simulink model "SWC_FDC_type"  (R2021b)
settings: Solver=FixedStepDiscrete  StartTime=0.0  StopTime=10.0  FixedStep=0.001  RelTol=1e-3
values from neighbouring files (symbols this model uses):
  C_TASK_5MS_S = (	C_TICK_TIME_S      	)    [vcu_local_hdr.m]
  DID_VCUKey = uint16(0x0202)    [vcu_local_hdr.m]
  DID_XWD = uint16(513)    [vcu_local_hdr.m]
  DIDLen_DKCKey = uint16(8)    [vcu_local_hdr.m]
  DIDLen_FoxPiBattSta = uint16(4)    [vcu_local_hdr.m]
  DIDLen_FoxPiBrakeSta = uint16(13)    [vcu_local_hdr.m]
  DIDLen_FoxPiButtonSta = uint16(2)    [vcu_local_hdr.m]
  DIDLen_FoxPiCtrlEnSw = uint16(1)    [vcu_local_hdr.m]
  DIDLen_FoxPiDrivingCtrl = uint16(21)    [vcu_local_hdr.m]
  DIDLen_FoxPiEPSSta = uint16(11)    [vcu_local_hdr.m]
  DIDLen_FoxPiLampCtrl = uint16(6)    [vcu_local_hdr.m]
  DIDLen_FoxPiLampSta = uint16(2)    [vcu_local_hdr.m]
  DIDLen_FoxPiMotionSta = uint16(13)    [vcu_local_hdr.m]
  DIDLen_FoxPiMotorSta = uint16(11)    [vcu_local_hdr.m]
  DIDLen_FoxPiPedalPos = uint16(3)    [vcu_local_hdr.m]
  DIDLen_FoxPiPTGUSSSw = uint16(1)    [vcu_local_hdr.m]
  DIDLen_FoxPiShifterAllow = uint16(3)    [vcu_local_hdr.m]
  DIDLen_FoxPiSwSta = uint16(2)    [vcu_local_hdr.m]
  DIDLen_FoxPiTPMSSta = uint16(13)    [vcu_local_hdr.m]
  DIDLen_FoxPiUSSDist = uint16(20)    [vcu_local_hdr.m]
  DIDLen_FoxPiUSSFaultSta = uint16(2)    [vcu_local_hdr.m]
  DIDLen_FoxPiWheelSpd = uint16(16)    [vcu_local_hdr.m]
  DIDNum_DKCKey = uint16(0x0202)    [vcu_local_hdr.m]
  DIDNum_FoxPiBattSta = uint16(0x100D)    [vcu_local_hdr.m]
  DIDNum_FoxPiBrakeSta = uint16(0x1003)    [vcu_local_hdr.m]
  DIDNum_FoxPiButtonSta = uint16(0x1006)    [vcu_local_hdr.m]
  DIDNum_FoxPiCtrlEnSw = uint16(0x1012)    [vcu_local_hdr.m]
  DIDNum_FoxPiDrivingCtrl = uint16(0x1001)    [vcu_local_hdr.m]
  DIDNum_FoxPiEPSSta = uint16(0x1005)    [vcu_local_hdr.m]
  DIDNum_FoxPiLampCtrl = uint16(0x100C)    [vcu_local_hdr.m]
  DIDNum_FoxPiLampSta = uint16(0x100B)    [vcu_local_hdr.m]
  DIDNum_FoxPiMotionSta = uint16(0x1002)    [vcu_local_hdr.m]
  DIDNum_FoxPiMotorSta = uint16(0x1010)    [vcu_local_hdr.m]
  DIDNum_FoxPiPedalPos = uint16(0x100F)    [vcu_local_hdr.m]
  DIDNum_FoxPiPTGUSSSw = uint16(0x1009)    [vcu_local_hdr.m]
  DIDNum_FoxPiShifterAllow = uint16(0x1011)    [vcu_local_hdr.m]
  DIDNum_FoxPiSwSta = uint16(0x100A)    [vcu_local_hdr.m]
  DIDNum_FoxPiTPMSSta = uint16(0x100E)    [vcu_local_hdr.m]
  DIDNum_FoxPiUSSDist = uint16(0x1007)    [vcu_local_hdr.m]
  DIDNum_FoxPiUSSFaultSta = uint16(0x1008)    [vcu_local_hdr.m]
  DIDNum_FoxPiWheelSpd = uint16(0x1004)    [vcu_local_hdr.m]
  DIDVCUKeyLength = uint16(8)    [vcu_local_hdr.m]
  DTC_10020B = Simulink.Parameter    [DTC_Constant_Definition.m]
  DTC_10020C = Simulink.Parameter    [DTC_Constant_Definition.m]
  DTC_10020D = Simulink.Parameter    [DTC_Constant_Definition.m]
  DTC_10020E = Simulink.Parameter    [DTC_Constant_Definition.m]
  DTC_100210 = Simulink.Parameter    [DTC_Constant_Definition.m]
  DTC_100211 = Simulink.Parameter    [DTC_Constant_Definition.m]
  DTC_100212 = Simulink.Parameter    [DTC_Constant_Definition.m]
  DTC_100213 = Simulink.Parameter    [DTC_Constant_Definition.m]
  DTC_100214 = Simulink.Parameter    [DTC_Constant_Definition.m]
  DTC_100215 = Simulink.Parameter    [DTC_Constant_Definition.m]
  DTC_100216 = Simulink.Parameter    [DTC_Constant_Definition.m]
  DTC_100217 = Simulink.Parameter    [DTC_Constant_Definition.m]
  DTC_100218 = Simulink.Parameter    [DTC_Constant_Definition.m]
  DTC_100219 = Simulink.Parameter    [DTC_Constant_Definition.m]
  DTC_10021A = Simulink.Parameter    [DTC_Constant_Definition.m]
  DTC_10021B = Simulink.Parameter    [DTC_Constant_Definition.m]
  DTC_10021C = Simulink.Parameter    [DTC_Constant_Definition.m]
  DTC_10021D = Simulink.Parameter    [DTC_Constant_Definition.m]
  DTC_10021E = Simulink.Parameter    [DTC_Constant_Definition.m]
  DTC_100220 = Simulink.Parameter    [DTC_Constant_Definition.m]
  DTC_100221 = Simulink.Parameter    [DTC_Constant_Definition.m]
  DTC_100223 = Simulink.Parameter    [DTC_Constant_Definition.m]
  DTC_100224 = Simulink.Parameter    [DTC_Constant_Definition.m]
  DTC_100225 = Simulink.Parameter    [DTC_Constant_Definition.m]
  DTC_100226 = Simulink.Parameter    [DTC_Constant_Definition.m]
  DTC_100227 = Simulink.Parameter    [DTC_Constant_Definition.m]
  DTC_100242 = Simulink.Parameter    [DTC_Constant_Definition.m]
  DTC_100243 = Simulink.Parameter    [DTC_Constant_Definition.m]
  DTC_100244 = Simulink.Parameter    [DTC_Constant_Definition.m]
  DTC_100247 = Simulink.Parameter    [DTC_Constant_Definition.m]
  DTC_100248 = Simulink.Parameter    [DTC_Constant_Definition.m]
  DTC_100249 = Simulink.Parameter    [DTC_Constant_Definition.m]
  DTC_100250 = Simulink.Parameter    [DTC_Constant_Definition.m]
  DTC_100251 = Simulink.Parameter    [DTC_Constant_Definition.m]
  DTC_100252 = Simulink.Parameter    [DTC_Constant_Definition.m]
  DTC_100A10 = Simulink.Parameter    [DTC_Constant_Definition.m]
  DTC_100A12 = Simulink.Parameter    [DTC_Constant_Definition.m]
  DTC_100A16 = Simulink.Parameter    [DTC_Constant_Definition.m]
  DTC_100A17 = Simulink.Parameter    [DTC_Constant_Definition.m]
  DTC_100A18 = Simulink.Parameter    [DTC_Constant_Definition.m]
  DTC_100A19 = Simulink.Parameter    [DTC_Constant_Definition.m]
  DTC_500B01 = Simulink.Parameter    [DTC_Constant_Definition.m]
  DTC_500B02 = Simulink.Parameter    [DTC_Constant_Definition.m]
  DTC_500B03 = Simulink.Parameter    [DTC_Constant_Definition.m]
  DTC_500B04 = Simulink.Parameter    [DTC_Constant_Definition.m]
  DTC_500B05 = Simulink.Parameter    [DTC_Constant_Definition.m]
  DTC_500B06 = Simulink.Parameter    [DTC_Constant_Definition.m]
  DTC_500B07 = Simulink.Parameter    [DTC_Constant_Definition.m]
  DTC_500B08 = Simulink.Parameter    [DTC_Constant_Definition.m]
  DTC_500B09 = Simulink.Parameter    [DTC_Constant_Definition.m]
  DTC_500B0A = Simulink.Parameter    [DTC_Constant_Definition.m]
  DTC_500B0B = Simulink.Parameter    [DTC_Constant_Definition.m]
  DTC_500B0C = Simulink.Parameter    [DTC_Constant_Definition.m]
  DTC_500B0D = Simulink.Parameter    [DTC_Constant_Definition.m]
  DTC_500B0E = Simulink.Parameter    [DTC_Constant_Definition.m]
  DTC_500B0F = Simulink.Parameter    [DTC_Constant_Definition.m]
  DTC_500B10 = Simulink.Parameter    [DTC_Constant_Definition.m]
  DTC_90021F = Simulink.Parameter    [DTC_Constant_Definition.m]
  DTC_90022F = Simulink.Parameter    [DTC_Constant_Definition.m]
  DTC_900253 = Simulink.Parameter    [DTC_Constant_Definition.m]
  DTC_900254 = Simulink.Parameter    [DTC_Constant_Definition.m]
  DTC_900301 = Simulink.Parameter    [DTC_Constant_Definition.m]
  DTC_900302 = Simulink.Parameter    [DTC_Constant_Definition.m]
  DTC_900303 = Simulink.Parameter    [DTC_Constant_Definition.m]
  DTC_900304 = Simulink.Parameter    [DTC_Constant_Definition.m]
  DTC_900305 = Simulink.Parameter    [DTC_Constant_Definition.m]
  DTC_900909 = Simulink.Parameter    [DTC_Constant_Definition.m]
  DTC_90090A = Simulink.Parameter    [DTC_Constant_Definition.m]
  DTC_90090B = Simulink.Parameter    [DTC_Constant_Definition.m]
  DTC_90090C = Simulink.Parameter    [DTC_Constant_Definition.m]
  DTC_90090D = Simulink.Parameter    [DTC_Constant_Definition.m]
  DTC_90090E = Simulink.Parameter    [DTC_Constant_Definition.m]
  DTC_90090F = Simulink.Parameter    [DTC_Constant_Definition.m]
  DTC_900910 = Simulink.Parameter    [DTC_Constant_Definition.m]
  DTC_900911 = Simulink.Parameter    [DTC_Constant_Definition.m]
  DTC_900912 = Simulink.Parameter    [DTC_Constant_Definition.m]
  DTC_900913 = Simulink.Parameter    [DTC_Constant_Definition.m]
  DTC_900914 = Simulink.Parameter    [DTC_Constant_Definition.m]
  ... (+54 more)
undefined symbols (not defined in the file or in its folder): f32_ApsOutVehSpdSig, KHAL_CANBusOffDebounce_cnt, KHAL_CANBusOffDebounce_s, KHAL_DKCDecryptEnable_flg_ovrdflg, KHAL_DKCDecryptEnable_flg_ovrdval, KHAL_RandomNumberY1_enum, KHAL_RandomNumberY2_enum, KHAL_RandomNumberY_ovrdflg, KHAL_TPMSRESBUTT_flg_ovrdflg, KHAL_TPMSRESBUTT_flg_ovrdval, KINP_ReadVinCode_flg, P_boolean, R_DIDWriteCDD_CSOP_DIDSet_DKCKey, R_DIDWriteCDD_CSOP_DIDSet_FoxPiBattSta, R_DIDWriteCDD_CSOP_DIDSet_FoxPiBrakeSta, R_DIDWriteCDD_CSOP_DIDSet_FoxPiButtonSta, R_DIDWriteCDD_CSOP_DIDSet_FoxPiCtrlEnSw, R_DIDWriteCDD_CSOP_DIDSet_FoxPiDrivingCtrl, R_DIDWriteCDD_CSOP_DIDSet_FoxPiEPSSta, R_DIDWriteCDD_CSOP_DIDSet_FoxPiLampCtrl, R_DIDWriteCDD_CSOP_DIDSet_FoxPiLampSta, R_DIDWriteCDD_CSOP_DIDSet_FoxPiMotionSta, R_DIDWriteCDD_CSOP_DIDSet_FoxPiMotorSta, R_DIDWriteCDD_CSOP_DIDSet_FoxPiPedalPos, R_DIDWriteCDD_CSOP_DIDSet_FoxPiPTGUSSSw, R_DIDWriteCDD_CSOP_DIDSet_FoxPiShifterAllow, R_DIDWriteCDD_CSOP_DIDSet_FoxPiSwSta, R_DIDWriteCDD_CSOP_DIDSet_FoxPiTPMSSta, R_DIDWriteCDD_CSOP_DIDSet_FoxPiUSSDist, R_DIDWriteCDD_CSOP_DIDSet_FoxPiUSSFaultSta, R_DIDWriteCDD_CSOP_DIDSet_FoxPiWheelSpd, R_E2E_CAN3_VCU1_CSOP_Write_CAN3_VCU1, R_E2E_CAN3_VCU1_toNIDEC_CSOP_Write_CAN3_VCU1_toNIDEC, R_E2E_CAN4_VCU1_CSOP_Write_CAN4_VCU1, R_FDCCDD_Inner_CSOP_FDC_AppCallSleep, R_HALIN_IMU_CSOP_IMUSetSta, R_HALINCDD_CSOP_PAS_Handler, R_HALINCDD_CSOP_ResetPedalZeroPosDone, R_HALINCDD_CSOP_TPMSSensorIDRegSetResults, R_HALINCDD_CSOP_UDS_Main, R_HALOUT_APS_CSOP_ApsOutput, R_HALOUTCDD_CSOP_AppNmStateReq, R_HALOUTCDD_CSOP_IVIReset, R_HALOUTCDD_CSOP_SetAcoreRebootCmdACK, R_HALOUTCDD_CSOP_SetSysPwrStat ... (+80)
libraries: FVT_lib x447, simulink x289, hcu_lib x19, hdlsllib x9, app x1, halin x1, halout x1, matrix_library x1, inp x1, outp x1
(part 7 of 15)

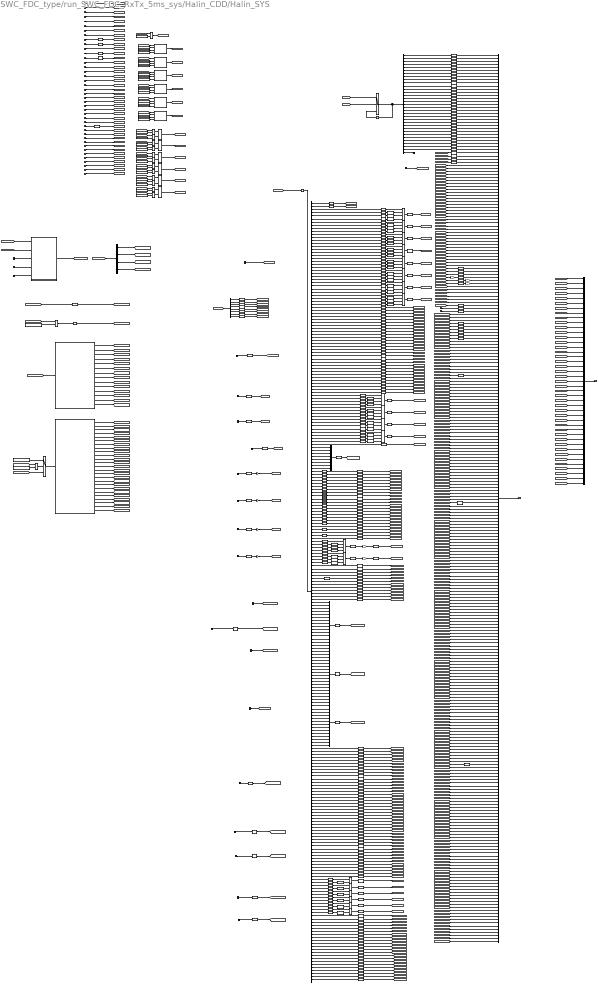
== system SWC_FDC_type/run_SWC_FDC_RxTx_5ms_sys/Halin_CDD/Halin_SYS ==
  note: Foxtron Pi
  note: CAN Bus Error
  note: CAN bus off debounce
  note: DID APS
  note: DID VCUKey
  note: DID BCM
  note: DID XWD
  GetSWID_status : Inport
  GetSWID_data : Inport  Port=2
  VHAL_AnyNMID_flg : Inport  Port=3
  VHAL_CurrentNmState_enum : Inport  Port=4
  VHAL_PwrReq_OTA_enum : Inport  Port=5
  VHAL_AllowMovThd_OTA_enum : Inport  Port=6
  VHAL_EvccAplusPwrUpReq_flg : Inport  Port=7
  VHAL_AcoreReadyToSlp_flg : Inport  Port=8
  VHAL_DidXWDSta_flg : Inport  Port=9
  VHAL_DidXWDData_enum : Inport  Port=10
  HAL_NvmReadData_raw : Inport  Port=11
  VHAL_DIDVCUKeyReadSta_flg : Inport  Port=12
  VHAL_GetDIDVCUKey_enum : Inport  Port=13
  VHAL_NvmProtectSta_flg : Inport  Port=14
  VHAL_AuxBattVolmV_100mV : Inport  Port=15
  VHAL_Pedal1Ref5V_raw : Inport  Port=16
  VHAL_Pedal2Ref5V_raw : Inport  Port=17
  VHAL_NetworkReqCalled_flg : Inport  Port=18
  VHAL_PmicBootReason_enum : Inport  Port=19
  VHAL_WisrBootReason_raw32 : Inport  Port=20
  BHAL_DIDGetData_raw : Inport  Port=21
  VHAL_AcoreRebootCmd_raw : Inport  Port=22
  VHAL_CAN1BusOff_raw : Inport  Port=23
  VHAL_CAN2BusOff_raw : Inport  Port=24
  VHAL_CAN3BusOff_raw : Inport  Port=25
  VHAL_CAN4BusOff_raw : Inport  Port=26
  VHAL_CAN5BusOff_raw : Inport  Port=27
  VHAL_CAN6BusOff_raw : Inport  Port=28
  VHAL_TPMSSensorIDRegSta_raw : Inport  Port=29
  VHAL_ResetPedalZeroPosReq_raw : Inport  Port=30
  VHAL_PmicBootPath_raw32 : Inport  Port=31
  VHAL_CAN1RxErrorCount_raw : Inport  Port=32
  VHAL_CAN1TxErrorCount_raw : Inport  Port=33
  VHAL_CAN2RxErrorCount_raw : Inport  Port=34
  VHAL_CAN2TxErrorCount_raw : Inport  Port=35
  VHAL_CAN3RxErrorCount_raw : Inport  Port=36
  VHAL_CAN3TxErrorCount_raw : Inport  Port=37
  VHAL_CAN4RxErrorCount_raw : Inport  Port=38
  VHAL_CAN4TxErrorCount_raw : Inport  Port=39
  VHAL_CAN5RxErrorCount_raw : Inport  Port=40
  VHAL_CAN5TxErrorCount_raw : Inport  Port=41
  VHAL_CAN6RxErrorCount_raw : Inport  Port=42
  VHAL_CAN6TxErrorCount_raw : Inport  Port=43
  AND : Logic  Inputs=1  AllPortsSameDT=off  OutDataTypeStr=boolean
  Bitwise OR{1..14} (14 alike) : simulink/Logic and Bit Operations/Bitwise Operator  logicop=OR  UseBitMask=off  NumInputPorts=4  BitMask=bin2dec('00000000000000000000')  BitMaskRealWorld=Stored Integer
  Bitwise OR{15..20} (6 alike) : simulink/Logic and Bit Operations/Bitwise Operator  logicop=OR  UseBitMask=off  NumInputPorts=2  BitMask=bin2dec('00000000000000000000')  BitMaskRealWorld=Stored Integer
  Bus Creator : BusCreator  Inputs=292  OutDataTypeStr=Bus: BHAL_SYS_outputs  NonVirtualBus=on
  Bus Creator4 : BusCreator  Inputs=43
  Bus Selector : BusSelector  OutputSignals=VHAL_DIDGetDKCKey_raw8,VHAL_DIDGetFoxPiDrivingCtrl_raw8,VHAL_DIDGetFoxPiLampCtrl_raw8,VHAL_DIDGetFoxPiCtrlEnSw_raw8
  Constant{,74..85} (13 alike) : Constant  Value=ZERO_INT
  Constant1 : Constant  Value=UINT8_MAX  OutDataTypeStr=uint8
  Constant2 : Constant  Value=ZERO_INT  OutDataTypeStr=uint8
  Constant4 : Constant  Value=UINT8_MAX  OutDataTypeStr=uint8
  Constant{56,58,60,62,65,71} (6 alike) : Constant  Value=C_TASK_5MS_S  OutDataTypeStr=single
  Constant{57,59,61,63,66,72} (6 alike) : Constant  Value=KHAL_CANBusOffDebounce_s  OutDataTypeStr=single
  Constant{64,67..70,73} (6 alike) : Constant  Value=KHAL_CANBusOffDebounce_cnt  OutDataTypeStr=single
  DIDGet_List : Subsystem
  Data Type Conversion{,3..30,33..44,49..55,98..104,106..107,109,112..121,127,133..135,139..141,143,164,187,190..195,207..210,212..234,236..237,239,241,243..250,252..255,274..282,285,288,290..293,296..297,299..302,814..822} (157 alike) : DataTypeConversion  OutDataTypeStr=uint8
  Data Type Conversion{1..2,31..32,45..48,56..57,105,108,110..111,122..126,128..132,136..138,142,180..185,188..189,200..201,211,235,238,240,242,251,283..284,287,294,298,318,823} (51 alike) : DataTypeConversion  OutDataTypeStr=boolean
  Data Type Conversion{58..97,144..163,169..178,186,295} (72 alike) : DataTypeConversion  OutDataTypeStr=uint32
  Data Type Conversion{165..166,168,179,196..199,202} (9 alike) : DataTypeConversion  OutDataTypeStr=single
  Data Type Conversion{167,256..273} (19 alike) : DataTypeConversion  OutDataTypeStr=uint16
  DebouncedFlg{,1..5} (6 alike) : hcu_lib/Basic_Blocks/DebouncedFlg
  Demux : Demux  Outputs=33
  Demux1 : Demux  Outputs=256
  Demux2 : Demux  Outputs=8
  Equal{,40..50} (12 alike) : RelationalOperator  Operator=>  OutDataTypeStr=boolean  RndMeth=Simplest
  Equal1 : RelationalOperator  Operator===  OutDataTypeStr=boolean  RndMeth=Simplest
  Equal2 : RelationalOperator  Operator===  OutDataTypeStr=boolean  RndMeth=Simplest
  FlashACForceOFF_Verify : Subsystem
  FlashACModeMem_Verify : Subsystem
  FlashAPMDoorControlSta : Subsystem
  FlashAirIntenZone1M_Verify : Subsystem
  FlashCCUSyncSts_Verify : Subsystem
  FlashCountAlarm_Verify : Subsystem
  FlashFaceM_Verify : Subsystem
  FlashFace_Verify : Subsystem
  FlashFootM_Verify : Subsystem
  FlashFoot_Verify : Subsystem
  FlashFrost_Verify : Subsystem
  FlashFuelDoorPos_Verify : Subsystem
  FlashMFRDNBrightReq_Verify : Subsystem
  FlashMFSWTri_Verify : Subsystem
  FlashMirrorFlodPos_Verify : Subsystem
  FlashRecAutoFlg_Verify : Subsystem
  FlashWiperFixMode_Verify : Subsystem
  Flashfdefog_Verify : Subsystem
  FlashsigRecircSt_Verify : Subsystem
  FlashsigSetTempZon1St_Verify : Subsystem
  FlashsigSetTempZon2StM_Verify : Subsystem
  FoxPiDrivingCtrl : Subsystem
  Gain : Gain  Gain=5/3788
  Gain1 : Gain  Gain=5/3788
  Gain2 : Gain  Gain=100
  Gain{4..7} (4 alike) : Gain  Gain=10
  Ground{,1..21} (22 alike) : Ground
  Logical Operator{14..19} (6 alike) : Logic  Operator=OR  AllPortsSameDT=off  OutDataTypeStr=boolean
  Multiply1 : Gain  Gain=1/10000
  Multiply2 : Gain  Gain=1/10000
  Mux : Mux  Inputs=8
  Mux1 : Mux  Inputs=16
  Mux2 : Mux  Inputs=16
  Mux3 : Mux  Inputs=16
  NotEqual : RelationalOperator  Operator=~=  OutDataTypeStr=boolean  RndMeth=Simplest
  Selector1 : Selector  InputPortWidth=256  IndexOptions=Index vector (dialog)  Indices=[1:256]  OutputSizes=1
  Shift Arithmetic{1,6,9,12,16,21,25,28..29,32,35..37,40,43..48} (20 alike) : ArithShift  BitShiftNumber=8  BitShiftDirection=Left
  Shift Arithmetic{2..3,7,10,13..14,17..18,22,26,30,33,38,41} (14 alike) : ArithShift  BitShiftNumber=16  BitShiftDirection=Left
  Shift Arithmetic{4..5,8,11,15,19..20,23..24,27,31,34,39,42} (14 alike) : ArithShift  BitShiftNumber=24  BitShiftDirection=Left
  Subsystem : Subsystem
  Switch : Switch  Criteria=u2 > Threshold
  Switch1 : Switch  Criteria=u2 ~= 0
  Terminator1 : Terminator
  Unit Delay1 : UnitDelay  SampleTime=-1  HasFrameUpgradeWarning=on
  BHAL_SYS_outputs : Outport  OutDataTypeStr=Bus:BHAL_SYS_outputs
  BHAL_SYSTPMS_outputs : Outport  Port=2
  wires:
  Data Type Conversion49/1 -> [VHAL_RFWheelPSW_raw8]  "VHAL_RFWheelPSW_raw8"
  Demux1/36 -> Data Type Conversion46/1
  Data Type Conversion91/1 -> Shift Arithmetic28/1
  Shift Arithmetic29/1 -> Bitwise OR5/2
  Shift Arithmetic14/1 -> Bitwise OR7/3
  Data Type Conversion73/1 -> Bitwise OR7/1
  Data Type Conversion86/1 -> Bitwise OR10/1
  Demux1/39 -> Data Type Conversion51/1
  Demux1/23 -> Data Type Conversion82/1
  Data Type Conversion71/1 -> Shift Arithmetic33/1
  Data Type Conversion48/1 -> [VHAL_RRSensorFail_flg]  "VHAL_RRSensorFail_flg"
  Data Type Conversion90/1 -> Bitwise OR11/1
  Shift Arithmetic18/1 -> Bitwise OR11/3
  [VHAL_EvccAplusPwrUpReq_flg] -> Data Type Conversion32/1
  Demux1/31 -> Data Type Conversion90/1
  Shift Arithmetic26/1 -> Bitwise OR10/3
  Shift Arithmetic32/1 -> Bitwise OR6/2
  Shift Arithmetic15/1 -> Bitwise OR7/4
  Demux1/30 -> Data Type Conversion89/1
  Data Type Conversion53/1 -> [VHAL_RFPindi_enum]  "VHAL_RFPindi_enum"
  Data Type Conversion95/1 -> [VHAL_FlashRFID_raw]  "VHAL_FlashRFID_raw"
  Demux1/7 -> Data Type Conversion65/1
  Ground/1 -> [VHAL_ReadFlashCorrect_flg]  "VHAL_ReadFlashCorrect_flg"
  Data Type Conversion92/1 -> Shift Arithmetic18/1
  Shift Arithmetic17/1 -> Bitwise OR8/3
  Shift Arithmetic16/1 -> Bitwise OR8/2
  Data Type Conversion54/1 -> [VHAL_FlashAntitheft_enum]  "VHAL_FlashAntitheft_enum"
  Shift Arithmetic22/1 -> Bitwise OR9/3
  Demux1/35 -> Data Type Conversion45/1
  Data Type Conversion78/1 -> [VHAL_FlashChkRFID_raw]  "VHAL_FlashChkRFID_raw"
  Shift Arithmetic21/1 -> Bitwise OR9/2
  Demux1/43 -> Data Type Conversion36/1
  Demux1/25 -> Data Type Conversion84/1
  Demux1/44 -> Data Type Conversion53/1
  Bus Creator/1 -> BHAL_SYS_outputs/1
  Demux1/45 -> Data Type Conversion35/1
  Demux1/14 -> Data Type Conversion72/1
  Demux1/29 -> Data Type Conversion88/1
  Demux1/24 -> Data Type Conversion83/1
  Data Type Conversion35/1 -> [VHAL_LRPindi_enum]  "VHAL_LRPindi_enum"
  Demux1/50 -> Data Type Conversion41/1
  GetSWID_status/1 -> [SYSOut]
  Data Type Conversion37/1 -> [VHAL_RRPindi_enum]  "VHAL_RRPindi_enum"
  Demux1/27 -> Data Type Conversion86/1
  Demux1/6 -> Data Type Conversion64/1
  Demux1/3 -> Data Type Conversion59/1
  Data Type Conversion41/1 -> [VHAL_RRP20_raw8]  "VHAL_RRP20_raw8"
  Data Type Conversion70/1 -> Shift Arithmetic32/1
  Data Type Conversion64/1 -> Shift Arithmetic24/1
  Demux1/9 -> Data Type Conversion67/1
  Shift Arithmetic30/1 -> Bitwise OR5/3
  Bitwise OR10/1 -> Data Type Conversion96/1
  Data Type Conversion45/1 -> [VHAL_LFSensorFail_flg]  "VHAL_LFSensorFail_flg"
  Demux1/32 -> Data Type Conversion91/1
  Switch1/1 -> Unit Delay1/1, Demux/1
  Demux1/46 -> Data Type Conversion37/1
  Shift Arithmetic19/1 -> Bitwise OR11/4
  Demux1/2 -> Data Type Conversion55/1
  Data Type Conversion108/1 -> [VHAL_DIDVCUKeyReadSta_flg]  "VHAL_DIDVCUKeyReadSta_flg"
  Data Type Conversion38/1 -> [VHAL_RFP20_raw8]  "VHAL_RFP20_raw8"
  [VHAL_AcoreReadyToSlp_flg] -> Data Type Conversion1/1
  Data Type Conversion74/1 -> Shift Arithmetic35/1
  Data Type Conversion60/1 -> Shift Arithmetic16/1
  Demux1/21 -> Data Type Conversion61/1
  Shift Arithmetic25/1 -> Bitwise OR10/2
  Data Type Conversion79/1 -> [VHAL_FlashChkLRID_raw]  "VHAL_FlashChkLRID_raw"
  Data Type Conversion81/1 -> Shift Arithmetic20/1
  Shift Arithmetic20/1 -> Bitwise OR8/4
  Demux1/11 -> Data Type Conversion69/1
  Data Type Conversion84/1 -> Shift Arithmetic22/1
  Demux1/62 -> Data Type Conversion106/1
  Data Type Conversion94/1 -> [VHAL_FlashLFID_raw]  "VHAL_FlashLFID_raw"
  Demux1/48 -> Data Type Conversion38/1
  Data Type Conversion98/1 -> [VHAL_RFWheelTemp_C]  "VHAL_RFWheelTemp_C"
  Shift Arithmetic12/1 -> Bitwise OR4/2
  Data Type Conversion83/1 -> Shift Arithmetic21/1
  Demux1/49 -> Data Type Conversion39/1
  Demux1/13 -> Data Type Conversion71/1
  Data Type Conversion69/1 -> Bitwise OR6/1
  Demux1/61 -> Data Type Conversion105/1
  Demux1/60 -> Data Type Conversion103/1
  Data Type Conversion104/1 -> [VHAL_Flashchkdatavalid_enum]  "VHAL_Flashchkdatavalid_enum"
  Demux1/59 -> Data Type Conversion104/1
  Bitwise OR7/1 -> Data Type Conversion80/1
  Data Type Conversion103/1 -> [VHAL_Flashdatavalid_enum]  "VHAL_Flashdatavalid_enum"
  Shift Arithmetic23/1 -> Bitwise OR9/4
  Demux1/58 -> Data Type Conversion101/1
  Demux1/20 -> Data Type Conversion60/1
  Data Type Conversion99/1 -> [VHAL_LRWheelTemp_C]  "VHAL_LRWheelTemp_C"
  Demux1/54 -> Data Type Conversion44/1
  Data Type Conversion82/1 -> Bitwise OR9/1
  Demux1/53 -> Data Type Conversion42/1
  Demux1/17 -> Data Type Conversion75/1
  Data Type Conversion96/1 -> [VHAL_FlashLRID_raw]  "VHAL_FlashLRID_raw"
  Demux1/8 -> Data Type Conversion66/1
  Demux1/37 -> Data Type Conversion47/1
  Demux1/34 -> Data Type Conversion93/1
  Demux1/10 -> Data Type Conversion68/1
  Data Type Conversion66/1 -> Shift Arithmetic29/1
  Shift Arithmetic24/1 -> Bitwise OR4/4
  Data Type Conversion50/1 -> [VHAL_LRWheelPSW_raw8]  "VHAL_LRWheelPSW_raw8"
  Data Type Conversion61/1 -> Shift Arithmetic17/1
  Bitwise OR9/1 -> Data Type Conversion95/1
  Data Type Conversion40/1 -> [VHAL_LFP20_raw8]  "VHAL_LFP20_raw8"
  Data Type Conversion46/1 -> [VHAL_RFSensorFail_flg]  "VHAL_RFSensorFail_flg"
  Data Type Conversion88/1 -> Shift Arithmetic26/1
  Data Type Conversion67/1 -> Shift Arithmetic30/1
  Data Type Conversion87/1 -> Shift Arithmetic25/1
  Demux1/1 -> Data Type Conversion54/1
  Data Type Conversion127/1 -> [VHAL_FlashAirIntenZone1M_enum]  "VHAL_FlashAirIntenZone1M_enum"
  Demux1/33 -> Data Type Conversion92/1
  Data Type Conversion106/1 -> [VHAL_unlearnSfailvalid_enum]  "VHAL_unlearnSfailvalid_enum"
  Demux1/52 -> Data Type Conversion102/1
  Data Type Conversion63/1 -> Shift Arithmetic13/1
  Data Type Conversion59/1 -> Bitwise OR4/1
  FlashFaceM_Verify/1(Out1) -> Data Type Conversion125/1
  Data Type Conversion93/1 -> Shift Arithmetic19/1
  Bitwise OR11/1 -> Data Type Conversion97/1
  VHAL_DIDVCUKeyReadSta_flg/1 -> Data Type Conversion108/1
  Bitwise OR5/1 -> Data Type Conversion78/1
  Data Type Conversion43/1 -> [VHAL_LFWheelPress_raw8]  "VHAL_LFWheelPress_raw8"
  Data Type Conversion62/1 -> Shift Arithmetic12/1
  Demux1/40 -> Data Type Conversion49/1
  Demux1/47 -> Data Type Conversion40/1
  Shift Arithmetic28/1 -> Bitwise OR11/2
  Data Type Conversion125/1 -> [VHAL_FlashFaceM_flg]  "VHAL_FlashFaceM_flg"
  Demux1/57 -> Data Type Conversion99/1
  FlashFootM_Verify/1(Out1) -> Data Type Conversion126/1
  Demux1/55 -> Data Type Conversion100/1
  Shift Arithmetic34/1 -> Bitwise OR6/4
  Demux1/63 -> Data Type Conversion107/1
  Data Type Conversion44/1 -> [VHAL_RRWheelPress_raw8]  "VHAL_RRWheelPress_raw8"
  FlashFoot_Verify/1(Out1) -> Data Type Conversion123/1
  Data Type Conversion100/1 -> [VHAL_LFWheelTemp_C]  "VHAL_LFWheelTemp_C"
  Data Type Conversion36/1 -> [VHAL_LFPindi_enum]  "VHAL_LFPindi_enum"
  Data Type Conversion76/1 -> Shift Arithmetic15/1
  [VHAL_PwrReq_OTA_enum] -> Data Type Conversion29/1
  Data Type Conversion55/1 -> [VHAL_DIDFlashXWDMode_raw8]  "VHAL_FlashDrivetrain_enum"
  Demux1/42 -> Data Type Conversion52/1
  Data Type Conversion121/1 -> [VHAL_FlashACModeMem_enum]  "VHAL_FlashACModeMem_enum"
  Data Type Conversion89/1 -> Shift Arithmetic27/1
  Data Type Conversion72/1 -> Shift Arithmetic34/1
  Data Type Conversion97/1 -> [VHAL_FlashRRID_raw]  "VHAL_FlashRRID_raw"
  VHAL_GetDIDVCUKey_enum/1 -> Data Type Conversion109/1
  Data Type Conversion85/1 -> Shift Arithmetic23/1
  Demux1/15 -> Data Type Conversion73/1
  [SYSbuffer] -> Switch1/1
  Data Type Conversion80/1 -> [VHAL_FlashChkRRID_raw]  "VHAL_FlashChkRRID_raw"
  Data Type Conversion123/1 -> [VHAL_FlashFoot_flg]  "VHAL_FlashFoot_flg"
  Demux1/56 -> Data Type Conversion98/1
  Data Type Conversion132/1 -> [VHAL_Flashfdefog_flg]  "VHAL_Flashfdefog_flg"
  Demux1/5 -> Data Type Conversion63/1
  Data Type Conversion101/1 -> [VHAL_RRWheelTemp_C]  "VHAL_RRWheelTemp_C"
  Data Type Conversion126/1 -> [VHAL_FlashFootM_flg]  "VHAL_FlashFootM_flg"
  Data Type Conversion65/1 -> Bitwise OR5/1
  Demux1/18 -> Data Type Conversion76/1
  Data Type Conversion102/1 -> [VHAL_RFWheelPress_raw8]  "VHAL_RFWheelPress_raw8"
  Data Type Conversion124/1 -> [VHAL_FlashFrost_flg]  "VHAL_FlashFrost_flg"
  Data Type Conversion68/1 -> Shift Arithmetic31/1
  [SYSOut] -> Switch1/2
  Unit Delay1/1 -> Switch1/3
  Demux1/16 -> Data Type Conversion74/1
  [VHAL_AllowMovThd_OTA_enum] -> Data Type Conversion30/1
  FlashFrost_Verify/1(Out1) -> Data Type Conversion124/1
  FlashACModeMem_Verify/1(Out1) -> Data Type Conversion121/1
  FlashsigRecircSt_Verify/1(Out1) -> Data Type Conversion130/1
  Demux1/26 -> Data Type Conversion85/1
  Shift Arithmetic35/1 -> Bitwise OR7/2
  Bitwise OR4/1 -> Data Type Conversion77/1
  Flashfdefog_Verify/1(Out1) -> Data Type Conversion132/1
  Shift Arithmetic33/1 -> Bitwise OR6/3
  FlashACForceOFF_Verify/1(Out1) -> Data Type Conversion129/1
  FlashCCUSyncSts_Verify/1(Out1) -> Data Type Conversion128/1
  FlashAirIntenZone1M_Verify/1(Out1) -> Data Type Conversion127/1
  FlashFace_Verify/1(Out1) -> Data Type Conversion122/1
  Data Type Conversion52/1 -> [VHAL_RRWheelPSW_raw8]  "VHAL_RRWheelPSW_raw8"
  Demux1/51 -> Data Type Conversion43/1
  Shift Arithmetic31/1 -> Bitwise OR5/4
  Data Type Conversion131/1 -> [VHAL_FlashRecAutoFlg_flg]  "VHAL_FlashRecAutoFlg_flg"
  FlashRecAutoFlg_Verify/1(Out1) -> Data Type Conversion131/1
  Bitwise OR8/1 -> Data Type Conversion94/1
  Data Type Conversion129/1 -> [VHAL_FlashACForceOFF_flg]  "VHAL_FlashACForceOFF_flg"
  Selector1/1 -> Demux1/1
  Data Type Conversion39/1 -> [VHAL_LRP20_raw8]  "VHAL_LRP20_raw8"
  Mux/1 -> Data Type Conversion120/1
  Data Type Conversion47/1 -> [VHAL_LRSensorFail_flg]  "VHAL_LRSensorFail_flg"
  Data Type Conversion42/1 -> [VHAL_LRWheelPress_raw8]  "VHAL_LRWheelPress_raw8"
  Demux1/38 -> Data Type Conversion48/1
  Data Type Conversion75/1 -> Shift Arithmetic14/1
  Data Type Conversion105/1 -> [VHAL_unlearnSfali_flg]  "VHAL_unlearnSfali_flg"
  Shift Arithmetic13/1 -> Bitwise OR4/3
  Data Type Conversion107/1 -> [VHAL_Prepresstempvalid_enum]  "VHAL_Prepresstempvalid_enum"
  Data Type Conversion120/1 -> [VHAL_DIDFlashDKCKey_raw8]
  Bitwise OR6/1 -> Data Type Conversion79/1
  Data Type Conversion58/1 -> Bitwise OR8/1
  Demux1/22 -> Data Type Conversion81/1
  Data Type Conversion130/1 -> [VHAL_FlashsigRecircSt_flg]  "VHAL_FlashsigRecircSt_flg"
  Data Type Conversion51/1 -> [VHAL_LFWheelPSW_raw8]  "VHAL_LFWheelPSW_raw8"
  Data Type Conversion77/1 -> [VHAL_FlashChkLFID_raw]  "VHAL_FlashChkLFID_raw"
  Data Type Conversion109/1 -> [VHAL_GetDIDVCUKey_raw]  "VHAL_GetDIDVCUKey_enum"
  Data Type Conversion122/1 -> [VHAL_FlashFace_flg]  "VHAL_FlashFace_flg"
  Shift Arithmetic27/1 -> Bitwise OR10/4
  Data Type Conversion128/1 -> [VHAL_FlashCCUSyncSts_flg]  "VHAL_FlashCCUSyncSts_flg"
  Demux1/4 -> Data Type Conversion62/1
  Demux1/41 -> Data Type Conversion50/1
  Demux1/12 -> Data Type Conversion70/1
  Demux1/28 -> Data Type Conversion87/1
  Demux1/19 -> Data Type Conversion58/1
  GetSWID_data/1 -> [SYSbuffer]
  VHAL_AcoreReadyToSlp_flg/1 -> [VHAL_AcoreReadyToSlp_flg]
  VHAL_AllowMovThd_OTA_enum/1 -> [VHAL_AllowMovThd_OTA_enum]
  VHAL_EvccAplusPwrUpReq_flg/1 -> [VHAL_EvccAplusPwrUpReq_flg]
  VHAL_PwrReq_OTA_enum/1 -> [VHAL_PwrReq_OTA_enum]
  VHAL_AnyNMID_flg/1 -> [VHAL_AnyNMID_flg]
  VHAL_CurrentNmState_enum/1 -> [VHAL_CurrentNmState_enum]
  Data Type Conversion2/1 -> [VHAL_DidXWDSta_flg]  "VHAL_DidXWDSta_flg"
  VHAL_DidXWDSta_flg/1 -> Data Type Conversion2/1
  Data Type Conversion3/1 -> [VHAL_DidXWDData_enum]  "VHAL_DidXWDData_enum"
  VHAL_DidXWDData_enum/1 -> Data Type Conversion3/1
  HAL_NvmReadData_raw/1 -> [HAL_NvmReadData_raw]
  [HAL_NvmReadData_raw] -> Selector1/1
  [VHAL_CurrentNmState_enum] -> Data Type Conversion33/1
  [VHAL_AnyNMID_flg] -> Data Type Conversion31/1
  Data Type Conversion134/1 -> [VHAL_FlashsigSetTempZon2StM_C]  "VHAL_FlashsigSetTempZon2StM_C"
  FlashMFSWTri_Verify/1(Out1) -> Data Type Conversion136/1
  Data Type Conversion142/1 -> [VHAL_FlashWiperFixMode_flg]  "VHAL_FlashWiperFixMode_flg"
  FlashWiperFixMode_Verify/1(Out1) -> Data Type Conversion142/1
  Data Type Conversion143/1 -> [VHAL_FlashIVIPTGUSStaSW_enum]  "VHAL_FlashIVIPTGUSStaSW_enum"
  FlashFuelDoorPos_Verify/1(Out1) -> Data Type Conversion138/1
  Demux1/111 -> Data Type Conversion143/1
  Data Type Conversion135/1 -> [VHAL_FlashCountAlarm_enum]  "VHAL_FlashCountAlarm_enum"
  Data Type Conversion141/1 -> [VHAL_FlashRoomLampMode_enum]  "VHAL_FlashRoomLampMode_enum"
  FlashMFRDNBrightReq_Verify/1(Out1) -> Data Type Conversion140/1
  Data Type Conversion139/1 -> [VHAL_FlashLockSetting_enum]  "VHAL_FlashLockSetting_enum"
  Data Type Conversion140/1 -> [VHAL_FlashMFRDNBrightReq_pct]  "VHAL_FlashMFRDNBrightReq_pct"
  Data Type Conversion138/1 -> [VHAL_FlashFuelDoorPos_flg]  "VHAL_FlashFuelDoorPos_flg"
  FlashsigSetTempZon2StM_Verify/1(Out1) -> Data Type Conversion134/1
  Data Type Conversion133/1 -> [VHAL_FlashsigSetTempZon1St_C]  "VHAL_FlashsigSetTempZon1St_C"
  Data Type Conversion136/1 -> [VHAL_FlashMFSWTri_flg]  "VHAL_FlashMFSWTri_flg"
  FlashMirrorFlodPos_Verify/1(Out1) -> Data Type Conversion137/1
  FlashsigSetTempZon1St_Verify/1(Out1) -> Data Type Conversion133/1
  Data Type Conversion137/1 -> [VHAL_FlashMirrorFlodPos_flg]  "VHAL_FlashMirrorFlodPos_flg"
  FlashCountAlarm_Verify/1(Out1) -> Data Type Conversion135/1
  [VHAL_LRP20_raw8] -> Bus Creator4/25
  [VHAL_LRWheelTemp_C] -> Bus Creator4/33
  [VHAL_Flashchkdatavalid_enum] -> Bus Creator4/9
  [VHAL_unlearnSfailvalid_enum] -> Bus Creator4/36
  [VHAL_RRPindi_enum] -> Bus Creator4/22
  [VHAL_FlashS3ID_raw] -> Bus Creator4/40
  [VHAL_LRSensorFail_flg] -> Bus Creator4/13
  [VHAL_FlashLFID_raw] -> Bus Creator4/5
  [VHAL_FlashChkRRID_raw] -> Bus Creator4/4
  [VHAL_FlashIDvaild_enum] -> Bus Creator4/42
  [VHAL_FlashChkRFID_raw] -> Bus Creator4/2
  [VHAL_LFWheelPSW_raw8] -> Bus Creator4/15
  [VHAL_RRWheelPSW_raw8] -> Bus Creator4/18
  [VHAL_RFWheelPress_raw8] -> Bus Creator4/28
  [VHAL_RRWheelPress_raw8] -> Bus Creator4/30
  [VHAL_FlashS2ID_raw] -> Bus Creator4/39
  [VHAL_unlearnSfali_flg] -> Bus Creator4/35
  [VHAL_LFWheelPress_raw8] -> Bus Creator4/27
  [VHAL_RRWheelTemp_C] -> Bus Creator4/34
  [VHAL_LRWheelPress_raw8] -> Bus Creator4/29
  [VHAL_Flashdatavalid_enum] -> Bus Creator4/10
  [VHAL_LFWheelTemp_C] -> Bus Creator4/31
  [VHAL_LFSensorFail_flg] -> Bus Creator4/11
  [VHAL_RRP20_raw8] -> Bus Creator4/26
  [VHAL_Prepresstempvalid_enum] -> Bus Creator4/37
  [VHAL_RFP20_raw8] -> Bus Creator4/24
  [VHAL_FlashRFID_raw] -> Bus Creator4/6
  [VHAL_FlashS4ID_raw] -> Bus Creator4/41
  [VHAL_LRPindi_enum] -> Bus Creator4/21
  Bus Creator4/1 -> BHAL_SYSTPMS_outputs/1
  [VHAL_LRWheelPSW_raw8] -> Bus Creator4/17
  [VHAL_RFPindi_enum] -> Bus Creator4/20
  [VHAL_FlashRRID_raw] -> Bus Creator4/8
  [VHAL_RFSensorFail_flg] -> Bus Creator4/12
  [VHAL_FlashChkLRID_raw] -> Bus Creator4/3
  [VHAL_RRSensorFail_flg] -> Bus Creator4/14
  [VHAL_RFWheelPSW_raw8] -> Bus Creator4/16
  [VHAL_LFP20_raw8] -> Bus Creator4/23
  [VHAL_RFWheelTemp_C] -> Bus Creator4/32
  [VHAL_FlashS1ID_raw] -> Bus Creator4/38
  [VHAL_FlashChkLFID_raw] -> Bus Creator4/1
  [VHAL_FlashLRID_raw] -> Bus Creator4/7
  [VHAL_LFPindi_enum] -> Bus Creator4/19
  Data Type Conversion150/1 -> Shift Arithmetic7/1
  Data Type Conversion156/1 -> Bitwise OR12/1
  Data Type Conversion147/1 -> Shift Arithmetic5/1
  Data Type Conversion151/1 -> Shift Arithmetic8/1
  Data Type Conversion161/1 -> [VHAL_FlashS2ID_raw]  "VHAL_FlashS2ID_raw"
  Demux1/66 -> Data Type Conversion146/1
  Demux1/64 -> Data Type Conversion144/1
  Data Type Conversion158/1 -> Shift Arithmetic3/1
  Demux1/79 -> Data Type Conversion159/1
  Data Type Conversion153/1 -> Shift Arithmetic9/1
  Shift Arithmetic8/1 -> Bitwise OR2/4
  Data Type Conversion144/1 -> Bitwise OR1/1
  Data Type Conversion154/1 -> Shift Arithmetic10/1
  Data Type Conversion159/1 -> Shift Arithmetic4/1
  Shift Arithmetic4/1 -> Bitwise OR12/4
  Demux1/70 -> Data Type Conversion150/1
  Demux1/71 -> Data Type Conversion151/1
  Data Type Conversion148/1 -> Bitwise OR2/1
  Demux1/80 -> Data Type Conversion164/1
  Shift Arithmetic5/1 -> Bitwise OR1/4
  Shift Arithmetic36/1 -> Bitwise OR12/2
  Demux1/68 -> Data Type Conversion148/1
  Shift Arithmetic1/1 -> Bitwise OR1/2
  Demux1/78 -> Data Type Conversion158/1
  Data Type Conversion146/1 -> Shift Arithmetic2/1
  Demux1/67 -> Data Type Conversion147/1
  Shift Arithmetic3/1 -> Bitwise OR12/3
  Data Type Conversion163/1 -> [VHAL_FlashS4ID_raw]  "VHAL_FlashS4ID_raw"
  Demux1/72 -> Data Type Conversion152/1
  Data Type Conversion155/1 -> Shift Arithmetic11/1
  Data Type Conversion160/1 -> [VHAL_FlashS1ID_raw]  "VHAL_FlashS1ID_raw"
  Demux1/69 -> Data Type Conversion149/1
  Bitwise OR12/1 -> Data Type Conversion163/1
  Data Type Conversion157/1 -> Shift Arithmetic36/1
  Bitwise OR1/1 -> Data Type Conversion160/1
  Shift Arithmetic10/1 -> Bitwise OR3/3
  Bitwise OR3/1 -> Data Type Conversion162/1
  Data Type Conversion162/1 -> [VHAL_FlashS3ID_raw]  "VHAL_FlashS3ID_raw"
  Shift Arithmetic7/1 -> Bitwise OR2/3
  Demux1/75 -> Data Type Conversion155/1
  Demux1/74 -> Data Type Conversion154/1
  Shift Arithmetic2/1 -> Bitwise OR1/3
  Data Type Conversion164/1 -> [VHAL_FlashIDvaild_enum]  "VHAL_FlashIDvalid_enum"
  Bitwise OR2/1 -> Data Type Conversion161/1
  Demux1/65 -> Data Type Conversion145/1
  Data Type Conversion149/1 -> Shift Arithmetic6/1
  Data Type Conversion145/1 -> Shift Arithmetic1/1
  Shift Arithmetic6/1 -> Bitwise OR2/2
  Shift Arithmetic11/1 -> Bitwise OR3/4
  Demux1/76 -> Data Type Conversion156/1
  Demux1/73 -> Data Type Conversion153/1
  Data Type Conversion152/1 -> Bitwise OR3/1
  Demux1/77 -> Data Type Conversion157/1
  Shift Arithmetic9/1 -> Bitwise OR3/2
  Demux1/81 -> Mux/1
  Demux1/82 -> Mux/2
  Demux1/83 -> Mux/3
  Demux1/84 -> Mux/4
  Demux1/85 -> Mux/5
  Demux1/86 -> Mux/6
  Demux1/87 -> Mux/7
  Demux1/88 -> Mux/8
  Demux1/89 -> FlashACModeMem_Verify/1(In1)
  Demux1/90 -> FlashFace_Verify/1(In1)
  Demux1/91 -> FlashFoot_Verify/1(In1)
  Demux1/92 -> FlashFrost_Verify/1(In1)
  Demux1/93 -> FlashFaceM_Verify/1(In1)
  Demux1/94 -> FlashFootM_Verify/1(In1)
  Demux1/95 -> FlashCCUSyncSts_Verify/1(In1)
  Demux1/96 -> FlashACForceOFF_Verify/1(In1)
  Demux1/97 -> FlashsigRecircSt_Verify/1(In1)
  Demux1/98 -> FlashRecAutoFlg_Verify/1(In1)
  Demux1/99 -> FlashAirIntenZone1M_Verify/1(In1)
  Demux1/100 -> Flashfdefog_Verify/1(In1)
  Demux1/101 -> FlashsigSetTempZon1St_Verify/1(In1)
  Demux1/102 -> FlashsigSetTempZon2StM_Verify/1(In1)
  Demux1/103 -> FlashCountAlarm_Verify/1(In1)
  Demux1/104 -> FlashMFSWTri_Verify/1(In1)
  Demux1/105 -> FlashMirrorFlodPos_Verify/1(In1)
  Demux1/106 -> FlashFuelDoorPos_Verify/1(In1)
  Demux1/108 -> FlashMFRDNBrightReq_Verify/1(In1)
  Demux1/110 -> FlashWiperFixMode_Verify/1(In1)
  [VHAL_NvmProtectSta_flg] -> Data Type Conversion56/1
  VHAL_NvmProtectSta_flg/1 -> [VHAL_NvmProtectSta_flg]
  Data Type Conversion166/1 -> Gain1/1
  Data Type Conversion165/1 -> Gain/1
  [VHAL_Pedal1Ref5V_raw] -> Data Type Conversion165/1
  [VHAL_Pedal2Ref5V_raw] -> Data Type Conversion166/1
  VHAL_AuxBattVolmV_100mV/1 -> [VHAL_AuxBattVolmV_100mV]
  VHAL_Pedal2Ref5V_raw/1 -> [VHAL_Pedal2Ref5V_raw]
  VHAL_Pedal1Ref5V_raw/1 -> [VHAL_Pedal1Ref5V_raw]
  [VHAL_AuxBattVolmV_100mV] -> Gain2/1
  Demux1/117 -> Data Type Conversion175/1
  Demux1/116 -> Data Type Conversion174/1
  Bitwise OR13/1 -> Data Type Conversion173/1
  Data Type Conversion177/1 -> Shift Arithmetic42/1
  Shift Arithmetic38/1 -> Bitwise OR13/3
  Demux1/114 -> Data Type Conversion171/1
  Shift Arithmetic41/1 -> Bitwise OR14/3
  Demux1/119 -> Data Type Conversion177/1
  Multiply2/1 -> Data Type Conversion168/1
  Data Type Conversion178/1 -> Multiply2/1
  Data Type Conversion175/1 -> Shift Arithmetic40/1
  Data Type Conversion173/1 -> Multiply1/1
  Shift Arithmetic42/1 -> Bitwise OR14/4
  Data Type Conversion176/1 -> Shift Arithmetic41/1
  Demux1/113 -> Data Type Conversion170/1
  Bitwise OR14/1 -> Data Type Conversion178/1
  Shift Arithmetic40/1 -> Bitwise OR14/2
  Data Type Conversion170/1 -> Shift Arithmetic37/1
  Data Type Conversion171/1 -> Shift Arithmetic38/1
  Data Type Conversion174/1 -> Bitwise OR14/1
  Data Type Conversion179/1 -> [VHAL_EAPS1MINMem_pct]  "VHAL_EAPS1MINMem_pct"
  Demux1/118 -> Data Type Conversion176/1
  Shift Arithmetic37/1 -> Bitwise OR13/2
  Demux1/115 -> Data Type Conversion172/1
  Demux1/112 -> Data Type Conversion169/1
  Data Type Conversion169/1 -> Bitwise OR13/1
  Shift Arithmetic39/1 -> Bitwise OR13/4
  Multiply1/1 -> Data Type Conversion179/1
  Data Type Conversion172/1 -> Shift Arithmetic39/1
  Data Type Conversion168/1 -> [VHAL_EAPS2MINMem_pct]  "VHAL_EAPS2MINMem_pct"
  Demux1/120 -> Data Type Conversion180/1
  Demux1/121 -> Data Type Conversion181/1
  Demux1/122 -> Data Type Conversion182/1
  Demux1/123 -> Data Type Conversion183/1
  Data Type Conversion180/1 -> [VHAL_FlashHoodSW_flg]  "VHAL_FlashHoodSW_flg"
  Data Type Conversion181/1 -> [VHAL_FlashTailgateSW_flg]  "VHAL_FlashTailgateSW_flg"
  Data Type Conversion182/1 -> [VHAL_FlashCTDLockSW_flg]  "VHAL_FlashCTDLockSW_flg"
  Data Type Conversion183/1 -> [VHAL_FlashTailgateHDSW_flg]  "VHAL_FlashTailgateHDSW_flg"
  VHAL_NetworkReqCalled_flg/1 -> [VHAL_NetworkReqCalled_flg]
  [VHAL_NetworkReqCalled_flg] -> Data Type Conversion184/1
  Gain2/1 -> Data Type Conversion167/1
  VHAL_PmicBootReason_enum/1 -> Data Type Conversion187/1
  VHAL_WisrBootReason_raw32/1 -> Data Type Conversion186/1
  Demux1/124 -> FlashAPMDoorControlSta/1(In1)
  FlashAPMDoorControlSta/1(Out1) -> Data Type Conversion185/1
  Data Type Conversion185/1 -> [VHAL_FlashAPMDoorControlSta_flg]  "VHAL_FlashAPMDoorControlSta_flg"
  BHAL_DIDGetData_raw/1 -> [BHAL_DIDGetData_raw]
  [BHAL_DIDOrigOutput_raw8] -> Bus Selector/1
  Bus Selector/1 -> [VHAL_DIDGetDKCKey_raw8]  "<VHAL_DIDGetDKCKey_raw8>"
  VHAL_AcoreRebootCmd_raw/1 -> [VHAL_AcoreRebootCmd_raw]  "VHAL_AcoreRebootCmd_raw"
  VHAL_CAN2BusOff_raw/1 -> [VHAL_CAN2BusOff_raw]  "VHAL_CAN2BusOff_raw"
  VHAL_CAN3BusOff_raw/1 -> [VHAL_CAN3BusOff_raw]  "VHAL_CAN3BusOff_raw"
  VHAL_CAN4BusOff_raw/1 -> [VHAL_CAN4BusOff_raw]  "VHAL_CAN4BusOff_raw"
  VHAL_CAN5BusOff_raw/1 -> [VHAL_CAN5BusOff_raw]  "VHAL_CAN5BusOff_raw"
  [VHAL_CAN1BusOff_flg] -> Data Type Conversion57/1
  [VHAL_CAN2BusOff_flg] -> Data Type Conversion110/1
  [VHAL_CAN3BusOff_flg] -> Data Type Conversion188/1
  [VHAL_CAN4BusOff_flg] -> Data Type Conversion111/1
  [VHAL_CAN5BusOff_flg] -> Data Type Conversion189/1
  [VHAL_AcoreRebootCmd_raw] -> NotEqual/1
  Constant/1 -> NotEqual/2
  NotEqual/1 -> [VHAL_AcoreRebootCmd_flg]
  Demux1/131 -> Data Type Conversion190/1
  Demux1/129 -> Data Type Conversion34/1
  Data Type Conversion34/1 -> [VHAL_DIDFlashTurnLampFRThreCurr_raw8]  "VHAL_DIDFlashTurnLampFRThreCurr_raw8"
  Demux1/130 -> Data Type Conversion192/1
  Demux1/128 -> Data Type Conversion191/1
  Demux1/127 -> Data Type Conversion193/1
  Demux1/126 -> Data Type Conversion195/1
  Data Type Conversion192/1 -> [VHAL_DIDFlashTurnLampRLThreCurr_raw8]  "VHAL_DIDFlashTurnLampRLThreCurr_raw8"
  Data Type Conversion195/1 -> [VHAL_DIDFlashDRLDis_raw8]  "VHAL_DIDFlashDRLDis_raw8"
  Data Type Conversion190/1 -> [VHAL_DIDFlashTurnLampRRThreCurr_raw8]  "VHAL_DIDFlashTurnLampRRThreCurr_raw8"
  Data Type Conversion193/1 -> [VHAL_DIDFlashFMHTimer_raw8]  "VHAL_DIDFlashFMHTimer_raw8"
  Demux1/125 -> Data Type Conversion194/1
  Data Type Conversion191/1 -> [VHAL_DIDFlashTurnLampFLThreCurr_raw8]  "VHAL_DIDFlashTurnLampFLThreCurr_raw8"
  Data Type Conversion194/1 -> [VHAL_DIDFlashAutoLock_raw8]  "VHAL_DIDFlashAutoLock_raw8"
  Demux1/132 -> Mux1/1
  Demux1/133 -> Mux1/2
  Demux1/134 -> Mux1/3
  Demux1/135 -> Mux1/4
  Demux1/136 -> Mux1/5
  Demux1/137 -> Mux1/6
  Demux1/138 -> Mux1/7
  Demux1/139 -> Mux1/8
  Demux1/140 -> Mux1/9
  Demux1/141 -> Mux1/10
  Demux1/142 -> Mux1/11
  Demux1/143 -> Mux1/12
  Demux1/144 -> Mux1/13
  Demux1/145 -> Mux1/14
  Demux1/146 -> Mux1/15
  Demux1/147 -> Mux1/16
  Mux1/1 -> Data Type Conversion208/1
  Data Type Conversion208/1 -> [VHAL_DIDFlashUSSConfig_raw8]  "VHAL_DIDFlashUSSConfig_raw8"
  Mux2/1 -> Data Type Conversion209/1
  Demux1/163 -> Mux2/16
  Demux1/162 -> Mux2/15
  Demux1/161 -> Mux2/14
  Demux1/160 -> Mux2/13
  Demux1/159 -> Mux2/12
  Demux1/158 -> Mux2/11
  Demux1/157 -> Mux2/10
  Demux1/156 -> Mux2/9
  Demux1/155 -> Mux2/8
  Demux1/154 -> Mux2/7
  Demux1/153 -> Mux2/6
  Demux1/152 -> Mux2/5
  Demux1/151 -> Mux2/4
  Demux1/150 -> Mux2/3
  Demux1/149 -> Mux2/2
  Demux1/148 -> Mux2/1
  Demux1/164 -> Mux3/1
  Demux1/165 -> Mux3/2
  Demux1/166 -> Mux3/3
  Demux1/167 -> Mux3/4
  Demux1/168 -> Mux3/5
  Demux1/169 -> Mux3/6
  Demux1/170 -> Mux3/7
  Demux1/171 -> Mux3/8
  Demux1/172 -> Mux3/9
  Demux1/173 -> Mux3/10
  Demux1/174 -> Mux3/11
  Demux1/175 -> Mux3/12
  Demux1/176 -> Mux3/13
  Demux1/177 -> Mux3/14
  Demux1/178 -> Mux3/15
  Demux1/179 -> Mux3/16
  Mux3/1 -> Data Type Conversion210/1
  Data Type Conversion209/1 -> [VHAL_DIDFlashTireSize_raw8]  "VHAL_DIDFlashTireSize_raw8"
  Data Type Conversion210/1 -> [VHAL_DIDFlashAPSFunConfig_raw8]  "VHAL_DIDFlashAPSFunConfig_raw8"
  Demux1/180 -> Data Type Conversion211/1
  Data Type Conversion211/1 -> [VHAL_FlashfUnlockSingle_flg]  "VHAL_FlashfUnlockSingle_flg"
  Demux1/181 -> Data Type Conversion212/1
  Data Type Conversion212/1 -> [VHAL_ReadRegenMode_enum]  "VHAL_ReadRegenMode_enum"
  [VHAL_FlashRegenMode_enum] -> Data Type Conversion213/1
  Data Type Conversion226/1 -> [VHAL_FlashAmbBrightnessSta1_enum]  "VHAL_FlashAmbBrightnessSta1_enum"
  Data Type Conversion228/1 -> [VHAL_FlashAmbBrightnessSta3_enum]  "VHAL_FlashAmbBrightnessSta3_enum"
  Demux1/189 -> Data Type Conversion221/1
  Demux1/187 -> Data Type Conversion220/1
  Data Type Conversion231/1 -> [VHAL_FlashAmbBrightnessSta7_enum]  "VHAL_FlashAmbBrightnessSta7_enum"
  Demux1/195 -> Data Type Conversion227/1
  Demux1/182 -> Data Type Conversion215/1
  Data Type Conversion230/1 -> [VHAL_FlashAmbBrightnessSta5_enum]  "VHAL_FlashAmbBrightnessSta5_enum"
  Demux1/185 -> Data Type Conversion218/1
  Data Type Conversion225/1 -> [VHAL_FlashAmbColorSta7_enum]  "VHAL_FlashAmbColorSta7_enum"
  Data Type Conversion215/1 -> [VHAL_FlashAmbFunEN_enum]  "VHAL_FlashAmbFunEN_enum"
  Demux1/186 -> Data Type Conversion219/1
  Data Type Conversion220/1 -> [VHAL_FlashAmbODAEN_enum]  "VHAL_FlashAmbODAEN_enum"
  Demux1/193 -> Data Type Conversion225/1
  Data Type Conversion222/1 -> [VHAL_FlashAmbColorSta3_enum]  "VHAL_FlashAmbColorSta3_enum"
  Demux1/199 -> Data Type Conversion231/1
  Data Type Conversion216/1 -> [VHAL_FlashAmbWelEN_enum]  "VHAL_FlashAmbWelEN_enum"
  Data Type Conversion218/1 -> [VHAL_FlashAmbLinkDriSta_enum]  "VHAL_FlashAmbLinkDriSta_enum"
  Demux1/191 -> Data Type Conversion223/1
  Demux1/192 -> Data Type Conversion224/1
  Demux1/194 -> Data Type Conversion226/1
  Demux1/196 -> Data Type Conversion228/1
  Data Type Conversion219/1 -> [VHAL_FlashAmbPwrWarnEN_enum]  "VHAL_FlashAmbPwrWarnEN_enum"
  Data Type Conversion214/1 -> [VHAL_FlashAmbColorSta1_enum]  "VHAL_FlashAmbColorSta1_enum"
  Data Type Conversion221/1 -> [VHAL_FlashAmbColorSta2_enum]  "VHAL_FlashAmbColorSta2_enum"
  Data Type Conversion223/1 -> [VHAL_FlashAmbColorSta4_enum]  "VHAL_FlashAmbColorSta4_enum"
  Demux1/197 -> Data Type Conversion229/1
  Demux1/183 -> Data Type Conversion216/1
  Demux1/190 -> Data Type Conversion222/1
  Data Type Conversion229/1 -> [VHAL_FlashAmbBrightnessSta4_enum]  "VHAL_FlashAmbBrightnessSta4_enum"
  Demux1/184 -> Data Type Conversion217/1
  Data Type Conversion227/1 -> [VHAL_FlashAmbBrightnessSta2_enum]  "VHAL_FlashAmbBrightnessSta2_enum"
  Demux1/188 -> Data Type Conversion214/1
  Demux1/198 -> Data Type Conversion230/1
  Data Type Conversion224/1 -> [VHAL_FlashAmbColorSta5_enum]  "VHAL_FlashAmbColorSta5_enum"
  Data Type Conversion217/1 -> [VHAL_FlashAmbDimEN_enum]  "VHAL_FlashAmbDimEN_enum"
  Demux1/200 -> Data Type Conversion232/1
  Demux1/201 -> Data Type Conversion233/1
  Data Type Conversion232/1 -> [VHAL_FlashTurnSwTSet123_enum]  "VHAL_FlashTurnSwTSet123_enum"
  Data Type Conversion233/1 -> [VHAL_FlashTurnSwTSet457_enum]  "VHAL_FlashTurnSwTSet457_enum"
  Data Type Conversion237/1 -> [VHAL_FlashDrEVentYSta_enum]  "VHAL_FlashDrEVentYSta_enum"
  Demux1/208 -> Data Type Conversion248/1
  Demux1/206 -> Data Type Conversion246/1
  Data Type Conversion241/1 -> [VHAL_FlashPsEVentYSta_enum]  "VHAL_FlashPsEVentYSta_enum"
  Data Type Conversion247/1 -> [VHAL_FlashPsEVentZSta_enum]  "VHAL_FlashPsEVentZSta_enum"
  Demux1/209 -> Data Type Conversion235/1
  Demux1/215 -> Data Type Conversion242/1
  Demux1/214 -> Data Type Conversion241/1
  Data Type Conversion234/1 -> [VHAL_FlashAirIntZ3Sta_enum]  "VHAL_FlashAirIntZ3Sta_enum"
  Data Type Conversion243/1 -> [VHAL_FlashPsEVentModeSta_enum]  "VHAL_FlashPsEVentModeSta_enum"
  Demux1/207 -> Data Type Conversion247/1
  Demux1/202 -> Data Type Conversion234/1
  Demux1/205 -> Data Type Conversion245/1
  Data Type Conversion238/1 -> [VHAL_FlashCLVentEN_flg]  "VHAL_FlashCLVentEN_flg"
  Demux1/204 -> Data Type Conversion244/1
  Demux1/210 -> Data Type Conversion237/1
  Demux1/213 -> Data Type Conversion240/1
  Data Type Conversion240/1 -> [VHAL_FlashPsVentEN_flg]  "VHAL_FlashPsVentEN_flg"
  Data Type Conversion242/1 -> [VHAL_FlashCRVentEN_flg]  "VHAL_FlashCRVentEN_flg"
  Demux1/203 -> Data Type Conversion243/1
  Demux1/216 -> Data Type Conversion236/1
  Data Type Conversion244/1 -> [VHAL_FlashDrEVentModeSta_enum]  "VHAL_FlashDrEVentModeSta_enum"
  Data Type Conversion248/1 -> [VHAL_FlashCREVentZSta_enum]  "VHAL_FlashCREVentZSta_enum"
  Data Type Conversion246/1 -> [VHAL_FlashCLEVentZSta_enum]  "VHAL_FlashCLEVentZSta_enum"
  Data Type Conversion235/1 -> [VHAL_FlashDrVentEN_flg]  "VHAL_FlashDrVentEN_flg"
  Data Type Conversion236/1 -> [VHAL_FlashCREVentYSta_enum]  "VHAL_FlashCREVentYSta_enum"
  Data Type Conversion239/1 -> [VHAL_FlashCLEVentYSta_enum]  "VHAL_FlashCLEVentYSta_enum"
  Demux1/211 -> Data Type Conversion238/1
  Demux1/212 -> Data Type Conversion239/1
  Data Type Conversion245/1 -> [VHAL_FlashDrEVentZSta_enum]  "VHAL_FlashDrEVentZSta_enum"
  Demux1/217 -> Data Type Conversion249/1
  Demux1/218 -> Data Type Conversion250/1
  Demux1/219 -> Data Type Conversion251/1
  Data Type Conversion249/1 -> [VHAL_FlashFGSAirIntSta_enum]  "VHAL_FlashFGSAirIntSta_enum"
  Data Type Conversion250/1 -> [VHAL_FlashFGSChSta_enum]  "VHAL_FlashFGSChSta_enum"
  Data Type Conversion251/1 -> [VHAL_FlashFGSIONSWSta_flg]  "VHAL_FlashFGSIONSWSta_flg"
  Demux1/107 -> Data Type Conversion139/1
  Demux1/220 -> Data Type Conversion252/1
  Demux1/222 -> Data Type Conversion255/1
  Demux1/221 -> Data Type Conversion253/1
  Data Type Conversion252/1 -> [VHAL_FlashWalkOutLkEN_enum]  "VHAL_FlashWalkOutLkEN_enum"
  Data Type Conversion253/1 -> [VHAL_FlashWalkInUnLkEN_enum]  "VHAL_FlashWalkInUnLkEN_enum"
  Data Type Conversion255/1 -> [VHAL_FlashFollowMeENFun_enum]  "VHAL_FlashFollowMeENFun_enum"
  Demux1/109 -> Data Type Conversion141/1
  [VHAL_TPMSSensorIDRegSta_raw] -> Bus Creator4/43
  VHAL_TPMSSensorIDRegSta_raw/1 -> [VHAL_TPMSSensorIDRegSta_raw]  "VHAL_TPMSSensorIDRegSta_raw"
  VHAL_ResetPedalZeroPosReq_raw/1 -> [VHAL_ResetPedalZeroPosReq_raw]
  [VHAL_ResetPedalZeroPosReq_raw] -> Data Type Conversion254/1
  Bitwise OR20/1 -> Data Type Conversion273/1
  Data Type Conversion274/1 -> [VHAL_FlashPTGOpenHeight12_enum]  "VHAL_FlashPTGOpenHeight12_enum"
  Shift Arithmetic45/1 -> Bitwise OR17/2
  Demux1/235 -> Data Type Conversion274/1
  Demux1/224 -> Data Type Conversion257/1
  Bitwise OR15/1 -> Data Type Conversion260/1
  Data Type Conversion275/1 -> [VHAL_FlashPTGOpenHeight34_enum]  "VHAL_FlashPTGOpenHeight34_enum"
  Shift Arithmetic48/1 -> Bitwise OR20/2
  Shift Arithmetic47/1 -> Bitwise OR19/2
  Data Type Conversion267/1 -> [VHAL_FlashPTGUserHeight4_cnt]  "VHAL_FlashPTGUserHeight4_cnt"
  Data Type Conversion276/1 -> [VHAL_FlashPTGOpenHeight57_enum]  "VHAL_FlashPTGOpenHeight57_enum"
  Demux1/237 -> Data Type Conversion276/1
  Data Type Conversion266/1 -> [VHAL_FlashPTGUserHeight3_cnt]  "VHAL_FlashPTGUserHeight3_cnt"
  Bitwise OR17/1 -> Data Type Conversion266/1
  Demux1/233 -> Data Type Conversion270/1
  Data Type Conversion272/1 -> [VHAL_FlashPTGUserHeight5_cnt]  "VHAL_FlashPTGUserHeight5_cnt"
  Bitwise OR16/1 -> Data Type Conversion261/1
  Data Type Conversion261/1 -> [VHAL_FlashPTGUserHeight2_cnt]  "VHAL_FlashPTGUserHeight2_cnt"
  Demux1/229 -> Data Type Conversion264/1
  Demux1/234 -> Data Type Conversion271/1
  Data Type Conversion262/1 -> Bitwise OR17/1
  Demux1/232 -> Data Type Conversion269/1
  Data Type Conversion270/1 -> Bitwise OR20/1
  Demux1/230 -> Data Type Conversion265/1
  Demux1/231 -> Data Type Conversion268/1
  Demux1/227 -> Data Type Conversion262/1
  Demux1/226 -> Data Type Conversion259/1
  Data Type Conversion271/1 -> Shift Arithmetic48/1
  Demux1/228 -> Data Type Conversion263/1
  Data Type Conversion265/1 -> Shift Arithmetic46/1
  Shift Arithmetic43/1 -> Bitwise OR15/2
  Shift Arithmetic44/1 -> Bitwise OR16/2
  Data Type Conversion260/1 -> [VHAL_FlashPTGUserHeight1_cnt]  "VHAL_FlashPTGUserHeight1_cnt"
  Bitwise OR19/1 -> Data Type Conversion272/1
  Demux1/236 -> Data Type Conversion275/1
  Data Type Conversion269/1 -> Shift Arithmetic47/1
  Data Type Conversion273/1 -> [VHAL_FlashPTGUserHeight7_cnt]  "VHAL_FlashPTGUserHeight7_cnt"
  Data Type Conversion263/1 -> Shift Arithmetic45/1
  Data Type Conversion258/1 -> Bitwise OR16/1
  Bitwise OR18/1 -> Data Type Conversion267/1
  Data Type Conversion259/1 -> Shift Arithmetic44/1
  Data Type Conversion257/1 -> Shift Arithmetic43/1
  Demux1/223 -> Data Type Conversion256/1
  Data Type Conversion268/1 -> Bitwise OR19/1
  Data Type Conversion256/1 -> Bitwise OR15/1
  Data Type Conversion264/1 -> Bitwise OR18/1
  Shift Arithmetic46/1 -> Bitwise OR18/2
  Demux1/225 -> Data Type Conversion258/1
  Data Type Conversion280/1 -> [VHAL_DIDFlashAutoWipHSpdEN_raw8]
  Data Type Conversion281/1 -> [VHAL_DIDFlashWipRLSCmdHoldFilter_raw8]
  Data Type Conversion282/1 -> [VHAL_DIDFlashWipRLSCmdCutFilter_raw8]
  Data Type Conversion291/1 -> [VHAL_FlashAutoUnlock_enum]  "VHAL_FlashAutoUnlock_enum"
  Data Type Conversion290/1 -> [VHAL_FlashAutoLock_enum]  "VHAL_FlashAutoLock_enum"
  Demux1/238 -> Data Type Conversion277/1
  Demux1/239 -> Data Type Conversion278/1
  Demux1/240 -> Data Type Conversion279/1
  Demux1/241 -> Data Type Conversion280/1
  Demux1/242 -> Data Type Conversion281/1
  Demux1/243 -> Data Type Conversion282/1
  Demux1/244 -> Data Type Conversion290/1
  Demux1/245 -> Data Type Conversion291/1
  Data Type Conversion277/1 -> [VHAL_FlashACCLevelSta12_enum]  "VHAL_FlashACCLevelSta12_enum"
  Data Type Conversion278/1 -> [VHAL_FlashACCLevelSta34_enum]  "VHAL_FlashACCLevelSta34_enum"
  Data Type Conversion279/1 -> [VHAL_FlashACCLevelSta57_enum]  "VHAL_FlashACCLevelSta57_enum"
  DebouncedFlg/1 -> [VHAL_CAN1BusOff_flg]
  [VHAL_CAN6BusOff_flg] -> Data Type Conversion294/1
  VHAL_CAN6BusOff_raw/1 -> [VHAL_CAN6BusOff_raw]  "VHAL_CAN6BusOff_raw"
  VHAL_PmicBootPath_raw32/1 -> Data Type Conversion295/1
  Data Type Conversion295/1 -> [VHAL_PmicBootPath_raw32]  "VHAL_PmicBootPath_raw32"
  Demux1/246 -> Data Type Conversion296/1
  Demux1/247 -> Data Type Conversion297/1
  Data Type Conversion296/1 -> [VHAL_FlashTPMModelVersion_raw]  "VHAL_FlashTPMModelVersion_raw"
  Data Type Conversion297/1 -> [VHAL_FlashTPMModelVersionChkSum_raw]  "VHAL_FlashTPMModelVersionChkSum_raw"
  [VHAL_VinCode_raw] -> Data Type Conversion814/1
  Demux1/251 -> Data Type Conversion818/1
  Demux1/253 -> Data Type Conversion820/1
  Data Type Conversion823/1 -> [VHAL_FlashAutoWipHSpdEN_flg]  "VHAL_FlashAutoWipHSpdEN_flg"
  Data Type Conversion815/1 -> [VHAL_FlashHMIKey1Func_enum]  "VHAL_FlashHMIKey1Func_enum"
  Demux1/248 -> Data Type Conversion815/1
  Data Type Conversion820/1 -> [VHAL_FlashHMIKey6Func_enum]  "VHAL_FlashHMIKey6Func_enum"
  Demux1/249 -> Data Type Conversion816/1
  Data Type Conversion822/1 -> [VHAL_FlashHMIKey8Func_enum]  "VHAL_FlashHMIKey8Func_enum"
  Data Type Conversion818/1 -> [VHAL_FlashHMIKey4Func_enum]  "VHAL_FlashHMIKey4Func_enum"
  Demux1/254 -> Data Type Conversion821/1
  Demux1/250 -> Data Type Conversion817/1
  Data Type Conversion819/1 -> [VHAL_FlashHMIKey5Func_enum]  "VHAL_FlashHMIKey5Func_enum"
  Demux1/255 -> Data Type Conversion822/1
  Demux1/252 -> Data Type Conversion819/1
  Demux1/256 -> Data Type Conversion823/1
  Data Type Conversion817/1 -> [VHAL_FlashHMIKey3Func_enum]  "VHAL_FlashHMIKey3Func_enum"
  Data Type Conversion821/1 -> [VHAL_FlashHMIKey7Func_enum]  "VHAL_FlashHMIKey7Func_enum"
  Data Type Conversion816/1 -> [VHAL_FlashHMIKey2Func_enum]  "VHAL_FlashHMIKey2Func_enum"
  Data Type Conversion254/1 -> Bus Creator/148  "VHAL_ResetPedalZeroPosReq_enum"
  Data Type Conversion213/1 -> Bus Creator/106  "VHAL_FlashRegenMode_enum"
  Gain1/1 -> Bus Creator/76  "VHAL_Pedal2Ref5V_V"
  Gain/1 -> Bus Creator/75  "VHAL_Pedal1Ref5V_V"
  Data Type Conversion294/1 -> Bus Creator/94  "VHAL_CAN6BusOff_flg"
  Data Type Conversion189/1 -> Bus Creator/93  "VHAL_CAN5BusOff_flg"
  Data Type Conversion111/1 -> Bus Creator/92  "VHAL_CAN4BusOff_flg"
  Data Type Conversion188/1 -> Bus Creator/91  "VHAL_CAN3BusOff_flg"
  Data Type Conversion110/1 -> Bus Creator/90  "VHAL_CAN2BusOff_flg"
  Data Type Conversion57/1 -> Bus Creator/89  "VHAL_CAN1BusOff_flg"
  [VHAL_FlashDrEVentZSta_enum] -> Bus Creator/130
  Data Type Conversion186/1 -> Bus Creator/85  "VHAL_WisrBootReason_raw32"
  [VHAL_FlashDrEVentModeSta_enum] -> Bus Creator/129
  [VHAL_FlashCLEVentZSta_enum] -> Bus Creator/131
  Data Type Conversion187/1 -> Bus Creator/84  "VHAL_PmicBootReason_enum"
  [VHAL_FlashPsEVentModeSta_enum] -> Bus Creator/128
  [VHAL_FlashPsEVentZSta_enum] -> Bus Creator/132
  Data Type Conversion184/1 -> Bus Creator/83  "VHAL_NetworkReqCalled_flg"
  [VHAL_FlashAirIntZ3Sta_enum] -> Bus Creator/127
  [VHAL_FlashCREVentZSta_enum] -> Bus Creator/133
  [VHAL_FlashTurnSwTSet457_enum] -> Bus Creator/126
  [VHAL_FlashDrVentEN_flg] -> Bus Creator/134
  [VHAL_FlashTurnSwTSet123_enum] -> Bus Creator/125
  [VHAL_FlashDrEVentYSta_enum] -> Bus Creator/135
  [VHAL_FlashAmbBrightnessSta7_enum] -> Bus Creator/124
  [VHAL_FlashCLVentEN_flg] -> Bus Creator/136
  [VHAL_FlashAmbBrightnessSta5_enum] -> Bus Creator/123
  [VHAL_FlashCLEVentYSta_enum] -> Bus Creator/137
  [VHAL_FlashAmbBrightnessSta4_enum] -> Bus Creator/122
  [VHAL_FlashPsVentEN_flg] -> Bus Creator/138
  [VHAL_FlashAmbBrightnessSta3_enum] -> Bus Creator/121
  [VHAL_FlashPsEVentYSta_enum] -> Bus Creator/139
  [VHAL_FlashAmbBrightnessSta2_enum] -> Bus Creator/120
  [VHAL_FlashCRVentEN_flg] -> Bus Creator/140
  [VHAL_FlashAmbBrightnessSta1_enum] -> Bus Creator/119
  [VHAL_FlashCREVentYSta_enum] -> Bus Creator/141
  Data Type Conversion167/1 -> Bus Creator/74  "VHAL_AuxBattVolmV_mV"
  [VHAL_FlashAmbColorSta7_enum] -> Bus Creator/118
  [VHAL_FlashFGSAirIntSta_enum] -> Bus Creator/142
  Data Type Conversion56/1 -> Bus Creator/73  "VHAL_NvmProtectSta_flg"
  [VHAL_FlashAmbColorSta5_enum] -> Bus Creator/117
  [VHAL_FlashFGSChSta_enum] -> Bus Creator/143
  Data Type Conversion33/1 -> Bus Creator/72  "VHAL_CurrentNmState_enum"
  [VHAL_FlashAmbColorSta4_enum] -> Bus Creator/116
  [VHAL_FlashFGSIONSWSta_flg] -> Bus Creator/144
  Data Type Conversion31/1 -> Bus Creator/71  "VHAL_AnyNMID_flg"
  [VHAL_FlashAmbColorSta3_enum] -> Bus Creator/115
  [VHAL_FlashWalkOutLkEN_enum] -> Bus Creator/145
  [VHAL_FlashAmbColorSta2_enum] -> Bus Creator/114
  [VHAL_FlashWalkInUnLkEN_enum] -> Bus Creator/146
  [VHAL_FlashAmbColorSta1_enum] -> Bus Creator/113
  [VHAL_FlashFollowMeENFun_enum] -> Bus Creator/147
  [VHAL_FlashAmbODAEN_enum] -> Bus Creator/112
  [VHAL_FlashAmbPwrWarnEN_enum] -> Bus Creator/111
  [VHAL_FlashPTGUserHeight1_cnt] -> Bus Creator/149
  [VHAL_FlashAmbLinkDriSta_enum] -> Bus Creator/110
  [VHAL_FlashPTGUserHeight2_cnt] -> Bus Creator/150
  [VHAL_FlashAmbDimEN_enum] -> Bus Creator/109
  [VHAL_FlashPTGUserHeight3_cnt] -> Bus Creator/151
  [VHAL_FlashAmbWelEN_enum] -> Bus Creator/108
  [VHAL_FlashPTGUserHeight4_cnt] -> Bus Creator/152
  [VHAL_FlashAmbFunEN_enum] -> Bus Creator/107
  [VHAL_FlashPTGUserHeight5_cnt] -> Bus Creator/153
  [VHAL_FlashPTGUserHeight7_cnt] -> Bus Creator/154
  [VHAL_FlashfUnlockSingle_flg] -> Bus Creator/105
  [VHAL_FlashPTGOpenHeight12_enum] -> Bus Creator/155
  [VHAL_APSFunConfig_raw8] -> Bus Creator/104  "VHAL_APSFunConfig_raw8"
  [VHAL_FlashPTGOpenHeight34_enum] -> Bus Creator/156
  [VHAL_TireSize_raw8] -> Bus Creator/103  "VHAL_TireSize_raw8"
  [VHAL_FlashPTGOpenHeight57_enum] -> Bus Creator/157
  [VHAL_USSConfig_raw8] -> Bus Creator/102  "VHAL_USSConfig_raw8"
  [VHAL_FlashACCLevelSta12_enum] -> Bus Creator/158
  [VHAL_DiagRRTC_mA] -> Bus Creator/101
  [VHAL_FlashACCLevelSta34_enum] -> Bus Creator/159
  [VHAL_DiagRLTC_mA] -> Bus Creator/100
  [VHAL_FlashACCLevelSta57_enum] -> Bus Creator/160
  [VHAL_DiagFRTC_mA] -> Bus Creator/99
  [VHAL_AutoWipHSpdEN_flg] -> Bus Creator/161
  [VHAL_DiagFLTC_mA] -> Bus Creator/98
  [VHAL_WipRLSCmdHoldEN_flg] -> Bus Creator/162
  [VHAL_DiagFMHT_s] -> Bus Creator/97
  [VHAL_WipRLSCmdHoldTime_s] -> Bus Creator/163
  [VHAL_DiagDRLOFF_flg] -> Bus Creator/96
  [VHAL_WipRLSCmdCutEN_flg] -> Bus Creator/164
  [VHAL_funAuto_flg] -> Bus Creator/95
  [VHAL_WipRLSCmdCutTime_s] -> Bus Creator/165
  [VHAL_FlashAutoLock_enum] -> Bus Creator/166
  [VHAL_FlashAutoUnlock_enum] -> Bus Creator/167
  [VHAL_PmicBootPath_raw32] -> Bus Creator/168
  [VHAL_FlashTPMModelVersion_raw] -> Bus Creator/169
  [VHAL_FlashTPMModelVersionChkSum_raw] -> Bus Creator/170
  [VHAL_FlashMILDIST_km] -> Bus Creator/171  "VHAL_FlashMILDIST_km"
  Data Type Conversion814/1 -> Bus Creator/234  "VHAL_VinCode_cnt"
  [VHAL_DIDGetDynoMode_flg] -> Bus Creator/88
  [VHAL_FlashWARMUPS_cnt] -> Bus Creator/172  "VHAL_FlashWARMUPS_cnt"
  [VHAL_AcoreRebootCmd_flg] -> Bus Creator/87  "VHAL_AcoreRebootCmd_flg"
  [VHAL_FlashCLRDIST_km] -> Bus Creator/173  "VHAL_FlashCLRDIST_km"
  [VHAL_FlashAPMDoorControlSta_flg] -> Bus Creator/86
  [VHAL_FlashMILTIME_min] -> Bus Creator/174  "VHAL_FlashMILTIME_min"
  [VHAL_FlashCLRTIME_min] -> Bus Creator/175  "VHAL_FlashCLRTIME_min"
  [VHAL_FlashNUMPSATRIPSFLTMEMCLR_cnt] -> Bus Creator/176  "VHAL_FlashNUMPSATRIPSFLTMEMCLR_cnt"
  [VHAL_FlashODOMETER_km] -> Bus Creator/177  "VHAL_FlashODOMETER_km"
  [VHAL_FlashPSAR_sec] -> Bus Creator/178  "VHAL_FlashPSAR_sec"
  [VHAL_FlashPSAL_sec] -> Bus Creator/179  "VHAL_FlashPSAL_sec"
  [VHAL_FlashIPSAR_sec] -> Bus Creator/180  "VHAL_FlashIPSAR_sec"
  [VHAL_FlashIPSAL_sec] -> Bus Creator/181  "VHAL_FlashIPSAL_sec"
  [VHAL_FlashCPSAR_sec] -> Bus Creator/182  "VHAL_FlashCPSAR_sec"
  [VHAL_FlashCPSAL_sec] -> Bus Creator/183  "VHAL_FlashCPSAL_sec"
  [VHAL_FlashHVBNAH_Ahr] -> Bus Creator/184  "VHAL_FlashHVBNAH_Ahr"
  [VHAL_FlashTailgateHDSW_flg] -> Bus Creator/82
  [VHAL_FlashHVBNE_kWh] -> Bus Creator/185  "VHAL_FlashHVBNE_kWh"
  [VHAL_FlashCTDLockSW_flg] -> Bus Creator/81
  [VHAL_FlashIGNCNTR_cnt] -> Bus Creator/186  "VHAL_FlashIGNCNTR_cnt"
  [VHAL_FlashTailgateSW_flg] -> Bus Creator/80
  [VHAL_FlashTNBCPSAR_Ahr] -> Bus Creator/187  "VHAL_FlashTNBCPSAR_Ahr"
  [VHAL_FlashHoodSW_flg] -> Bus Creator/79
  [VHAL_FlashTNBCPSAL_Ahr] -> Bus Creator/188  "VHAL_FlashTNBCPSAL_Ahr"
  [VHAL_FlashTNECPSAR_kWh] -> Bus Creator/189  "VHAL_FlashTNECPSAR_kWh"
  [VHAL_EAPS2MINMem_pct] -> Bus Creator/78
  [VHAL_FlashTNECPSAL_kWh] -> Bus Creator/190  "VHAL_FlashTNECPSAL_kWh"
  [VHAL_EAPS1MINMem_pct] -> Bus Creator/77
  [VHAL_FlashTEBPSAR_kWh] -> Bus Creator/191  "VHAL_FlashTEBPSAR_kWh"
  [VHAL_FlashTEBPSAL_kWh] -> Bus Creator/192  "VHAL_FlashTEBPSAL_kWh"
  [VHAL_FlashTGEOVCR_kWh] -> Bus Creator/193  "VHAL_FlashTGEOVCR_kWh"
  [VHAL_FlashTGEOVCL_kWh] -> Bus Creator/194  "VHAL_FlashTGEOVCL_kWh"
  [VHAL_FlashGECHGOVCDCR_kWh] -> Bus Creator/195  "VHAL_FlashGECHGOVCDCR_kWh"
  [VHAL_FlashGECHGOVCDCL_kWh] -> Bus Creator/196  "VHAL_FlashGECHGOVCDCL_kWh"
  [VHAL_FlashGECHGOVCACR_kWh] -> Bus Creator/197  "VHAL_FlashGECHGOVCACR_kWh"
  [VHAL_FlashGECHGOVCACL_kWh] -> Bus Creator/198  "VHAL_FlashGECHGOVCACL_kWh"
  [VHAL_FlashRESSV2XENNONPSAR_kWh] -> Bus Creator/199  "VHAL_FlashRESSV2XENNONPSAR_kWh"
  [VHAL_FlashIVIPTGUSStaSW_enum] -> Bus Creator/70
  [VHAL_FlashRESSV2XENNONPSAL_kWh] -> Bus Creator/200  "VHAL_FlashRESSV2XENNONPSAL_kWh"
  [VHAL_FlashWiperFixMode_flg] -> Bus Creator/69
  [VHAL_FlashPKERNumerator_kphsqr] -> Bus Creator/201  "VHAL_FlashPKERNumerator_kphsqr"
  Data Type Conversion32/1 -> Bus Creator/36  "VHAL_EvccAplusPwrUpReq_flg"
  [VHAL_FlashRoomLampMode_enum] -> Bus Creator/68
  [VHAL_FlashPKELNumerator_kphsqr] -> Bus Creator/202  "VHAL_FlashPKELNumerator_kphsqr"
  Data Type Conversion30/1 -> Bus Creator/35  "VHAL_AllowMovThd_OTA_enum"
  [VHAL_FlashMFRDNBrightReq_pct] -> Bus Creator/67
  [VHAL_FlashResetCDEODTR_km] -> Bus Creator/203  "VHAL_FlashResetCDEODTR_km"
  Data Type Conversion29/1 -> Bus Creator/34  "VHAL_PwrReq_OTA_enum"
  [VHAL_FlashLockSetting_enum] -> Bus Creator/66
  [VHAL_FlashAvgBattTempPSAR_C] -> Bus Creator/204  "VHAL_FlashAvgBattTempPSAR_C"
  Data Type Conversion1/1 -> Bus Creator/33  "VHAL_AcoreReadyToSlp_flg"
  [VHAL_FlashFuelDoorPos_flg] -> Bus Creator/65
  [VHAL_FlashAvgBattTempPSAL_C] -> Bus Creator/205  "VHAL_FlashAvgBattTempPSAL_C"
  Data Type Conversion28/1 -> Bus Creator/32  "VHAL_SHA8_cnt"
  [VHAL_FlashMirrorFlodPos_flg] -> Bus Creator/64
  [VHAL_FlashAvgBattTempOVCR_C] -> Bus Creator/206  "VHAL_FlashAvgBattTempOVCR_C"
  Data Type Conversion27/1 -> Bus Creator/31  "VHAL_SHA7_cnt"
  [VHAL_FlashMFSWTri_flg] -> Bus Creator/63
  [VHAL_FlashAvgBattTempOVCL_C] -> Bus Creator/207  "VHAL_FlashAvgBattTempOVCL_C"
  Data Type Conversion26/1 -> Bus Creator/30  "VHAL_SHA6_cnt"
  [VHAL_FlashCountAlarm_enum] -> Bus Creator/62
  [VHAL_FlashAvgBattTempOFFR_C] -> Bus Creator/208  "VHAL_FlashAvgBattTempOFFR_C"
  Data Type Conversion25/1 -> Bus Creator/29  "VHAL_SHA5_cnt"
  [VHAL_FlashsigSetTempZon2StM_C] -> Bus Creator/61
  [VHAL_FlashAvgBattTempOFFL_C] -> Bus Creator/209  "VHAL_FlashAvgBattTempOFFL_C"
  Data Type Conversion24/1 -> Bus Creator/28  "VHAL_SHA4_cnt"
  [VHAL_FlashsigSetTempZon1St_C] -> Bus Creator/60
  [VHAL_FlashQTYPSATRIPSR_cnt] -> Bus Creator/210  "VHAL_FlashQTYPSATRIPSR_cnt"
  Data Type Conversion23/1 -> Bus Creator/27  "VHAL_SHA3_cnt"
  [VHAL_Flashfdefog_flg] -> Bus Creator/59
  [VHAL_FlashQTYPSATRIPSL_cnt] -> Bus Creator/211  "VHAL_FlashQTYPSATRIPSL_cnt"
  Data Type Conversion22/1 -> Bus Creator/26  "VHAL_SHA2_cnt"
  [VHAL_FlashAirIntenZone1M_enum] -> Bus Creator/58
  [VHAL_FlashRESSCNTDODRNGR_cnt] -> Bus Creator/212  "VHAL_FlashRESSCNTDODRNGR_cnt"
  Data Type Conversion21/1 -> Bus Creator/25  "VHAL_SHA1_cnt"
  [VHAL_FlashRecAutoFlg_flg] -> Bus Creator/57
  [VHAL_FlashRESSCNTDODRNGL_cnt] -> Bus Creator/213  "VHAL_FlashRESSCNTDODRNGL_cnt"
  Data Type Conversion20/1 -> Bus Creator/24  "VHAL_Dash2_cnt"
  [VHAL_FlashsigRecircSt_flg] -> Bus Creator/56
  [VHAL_FlashETMATOER_kWh] -> Bus Creator/214  "VHAL_FlashETMATOER_kWh"
  Data Type Conversion19/1 -> Bus Creator/23  "VHAL_Change2_cnt"
  [VHAL_FlashACForceOFF_flg] -> Bus Creator/55
  [VHAL_FlashETMATOEL_kWh] -> Bus Creator/215  "VHAL_FlashETMATOEL_kWh"
  Data Type Conversion18/1 -> Bus Creator/22  "VHAL_Change1_cnt"
  [VHAL_FlashCCUSyncSts_flg] -> Bus Creator/54
  [VHAL_FlashETMBTOER_kWh] -> Bus Creator/216  "VHAL_FlashETMBTOER_kWh"
  Data Type Conversion292/1 -> Bus Creator/21  "VHAL_Dash1_cnt"
  [VHAL_FlashFootM_flg] -> Bus Creator/53
  [VHAL_FlashETMBTOEL_kWh] -> Bus Creator/217  "VHAL_FlashETMBTOEL_kWh"
  [VHAL_FlashFaceM_flg] -> Bus Creator/52
  [VHAL_FlashRESSTIMESOCPSARNGR_s] -> Bus Creator/218  "VHAL_FlashRESSTIMESOCPSARNGR_s"
  Data Type Conversion299/1 -> Bus Creator/17  "VHAL_DrivingMode_cnt"
  [VHAL_FlashFrost_flg] -> Bus Creator/51
  [VHAL_FlashRESSTIMESOCPSARNGL_s] -> Bus Creator/219  "VHAL_FlashRESSTIMESOCPSARNGL_s"
  Data Type Conversion293/1 -> Bus Creator/16  "VHAL_ECUGen2_cnt"
  [VHAL_FlashFoot_flg] -> Bus Creator/50
  [VHAL_FlashRESSTIMESOCCHGRNGR_s] -> Bus Creator/220  "VHAL_FlashRESSTIMESOCCHGRNGR_s"
  Data Type Conversion17/1 -> Bus Creator/15  "VHAL_ECUGen1_cnt"
  [VHAL_FlashFace_flg] -> Bus Creator/49
  [VHAL_FlashRESSTIMESOCCHGRNGL_s] -> Bus Creator/221  "VHAL_FlashRESSTIMESOCCHGRNGL_s"
  Data Type Conversion16/1 -> Bus Creator/14  "VHAL_Variation_cnt"
  [VHAL_FlashACModeMem_enum] -> Bus Creator/48
  [VHAL_FlashRESSTIMESOCOFFRNGR_s] -> Bus Creator/222  "VHAL_FlashRESSTIMESOCOFFRNGR_s"
  Data Type Conversion15/1 -> Bus Creator/13  "VHAL_Country2_cnt"
  [VHAL_RandomnumberY_raw8] -> Bus Creator/47
  [VHAL_FlashRESSTIMESOCOFFRNGL_s] -> Bus Creator/223  "VHAL_FlashRESSTIMESOCOFFRNGL_s"
  Data Type Conversion14/1 -> Bus Creator/12  "VHAL_Country1_cnt"
  [VHAL_RandomnumberY_raw7] -> Bus Creator/46
  [VHAL_FlashMAXBATTEMPL_C] -> Bus Creator/224  "VHAL_FlashMAXBATTEMPL_C"
  Data Type Conversion13/1 -> Bus Creator/11  "VHAL_Patch2_cnt"
  [VHAL_RandomnumberY_raw6] -> Bus Creator/45
  [VHAL_FlashMINBATTEMPL_C] -> Bus Creator/225  "VHAL_FlashMINBATTEMPL_C"
  Data Type Conversion12/1 -> Bus Creator/10  "VHAL_Patch1_cnt"
  [VHAL_RandomnumberY_raw5] -> Bus Creator/44
  [VHAL_FlashAVGBATTEMPL_sec] -> Bus Creator/226  "VHAL_FlashAVGBATTEMPL_sec"
  Data Type Conversion11/1 -> Bus Creator/9  "VHAL_Minor2_cnt"
  [VHAL_RandomnumberY_raw4] -> Bus Creator/43
  [VHAL_FlashAVGBATTEMPL_C] -> Bus Creator/227  "VHAL_FlashAVGBATTEMPL_C"
  Data Type Conversion10/1 -> Bus Creator/8  "VHAL_Minor1_cnt"
  [VHAL_RandomnumberY_raw3] -> Bus Creator/42
  [VHAL_FlashBattTempPSAR_sec] -> Bus Creator/228  "VHAL_FlashBattTempPSAR_sec"
  Data Type Conversion9/1 -> Bus Creator/7  "VHAL_Major2_cnt"
  [VHAL_RandomnumberY_raw2] -> Bus Creator/41
  [VHAL_FlashBattTempPSAL_sec] -> Bus Creator/229  "VHAL_FlashBattTempPSAL_sec"
  Data Type Conversion8/1 -> Bus Creator/6  "VHAL_Major1_cnt"
  [VHAL_RandomnumberY_raw1] -> Bus Creator/40
  [VHAL_FlashOVCR_sec] -> Bus Creator/230  "VHAL_FlashOVCR_sec"
  Data Type Conversion7/1 -> Bus Creator/5  "VHAL_ECU2_cnt"
  [VHAL_FlashAntitheft_enum] -> Bus Creator/39
  [VHAL_FlashOVCL_sec] -> Bus Creator/231  "VHAL_FlashOVCL_sec"
  Data Type Conversion6/1 -> Bus Creator/4  "VHAL_ECU1_cnt"
  [VHAL_ReadFlashCorrect_flg] -> Bus Creator/38
  [VHAL_FlashOFFR_sec] -> Bus Creator/232  "VHAL_FlashOFFR_sec"
  Data Type Conversion5/1 -> Bus Creator/3  "VHAL_CarModel3_cnt"
  [VHAL_DrivetrainSelect_enum] -> Bus Creator/37
  [VHAL_FlashOFFL_sec] -> Bus Creator/233  "VHAL_FlashOFFL_sec"
  Data Type Conversion4/1 -> Bus Creator/2  "VHAL_CarModel2_cnt"
  Data Type Conversion/1 -> Bus Creator/1  "VHAL_CarMode1_cnt"
  [VHAL_FlashHMIKey1Func_enum] -> Bus Creator/235  "VHAL_FlashHMIKey1Func_enum"
  [VHAL_FlashHMIKey2Func_enum] -> Bus Creator/236  "VHAL_FlashHMIKey2Func_enum"
  [VHAL_FlashHMIKey3Func_enum] -> Bus Creator/237  "VHAL_FlashHMIKey3Func_enum"
  [VHAL_FlashHMIKey4Func_enum] -> Bus Creator/238  "VHAL_FlashHMIKey4Func_enum"
  [VHAL_FlashHMIKey5Func_enum] -> Bus Creator/239  "VHAL_FlashHMIKey5Func_enum"
  [VHAL_FlashHMIKey6Func_enum] -> Bus Creator/240  "VHAL_FlashHMIKey6Func_enum"
  [VHAL_FlashHMIKey7Func_enum] -> Bus Creator/241  "VHAL_FlashHMIKey7Func_enum"
  [VHAL_FlashHMIKey8Func_enum] -> Bus Creator/242  "VHAL_FlashHMIKey8Func_enum"
  [VHAL_FlashAutoWipHSpdEN_flg] -> Bus Creator/243  "VHAL_FlashAutoWipHSpdEN_flg"
  [VHAL_FlashDIDModelVersion_raw] -> Bus Creator/244  "VHAL_FlashDIDModelVersion_raw"
  [VHAL_FlashDIDModelVersionChkSum_raw] -> Bus Creator/245  "VHAL_FlashDIDModelVersionChkSum_raw"
  Demux/33 -> Terminator1/1
  Demux/1 -> Data Type Conversion/1
  Demux/2 -> Data Type Conversion4/1
  Demux/3 -> Data Type Conversion5/1
  Demux/4 -> Data Type Conversion6/1
  Demux/5 -> Data Type Conversion7/1
  Demux/6 -> Data Type Conversion8/1
  Demux/7 -> Data Type Conversion9/1
  Demux/8 -> Data Type Conversion10/1
  Demux/9 -> Data Type Conversion11/1
  Demux/10 -> Data Type Conversion12/1
  Demux/11 -> Data Type Conversion13/1
  Demux/12 -> Data Type Conversion14/1
  Demux/13 -> Data Type Conversion15/1
  Demux/14 -> Data Type Conversion16/1
  Demux/15 -> Data Type Conversion17/1
  Demux/16 -> Data Type Conversion293/1
  Demux/17 -> Data Type Conversion299/1
  Demux/18 -> Data Type Conversion300/1
  Demux/19 -> Data Type Conversion302/1
  Demux/20 -> Data Type Conversion301/1
  Demux/21 -> Data Type Conversion292/1
  Demux/22 -> Data Type Conversion18/1
  Demux/23 -> Data Type Conversion19/1
  Demux/24 -> Data Type Conversion20/1
  Demux/25 -> Data Type Conversion21/1
  Demux/26 -> Data Type Conversion22/1
  Demux/27 -> Data Type Conversion23/1
  Demux/28 -> Data Type Conversion24/1
  Demux/29 -> Data Type Conversion25/1
  Demux/30 -> Data Type Conversion26/1
  Demux/31 -> Data Type Conversion27/1
  Demux/32 -> Data Type Conversion28/1
  Data Type Conversion301/1 -> Bus Creator/20  "VHAL_Var5_cnt"
  Data Type Conversion302/1 -> Bus Creator/19  "VHAL_Var4_cnt"
  Data Type Conversion300/1 -> Bus Creator/18  "VHAL_ModelYear_cnt"
  [VHAL_CAN1BusOff_raw] -> DebouncedFlg/1
  Constant56/1 -> DebouncedFlg/2
  Constant57/1 -> DebouncedFlg/3
  Constant68/1 -> DebouncedFlg/4
  Constant69/1 -> DebouncedFlg1/4
  Constant59/1 -> DebouncedFlg1/3
  Constant58/1 -> DebouncedFlg1/2
  DebouncedFlg1/1 -> [VHAL_CAN2BusOff_flg]
  [VHAL_CAN2BusOff_raw] -> DebouncedFlg1/1
  DebouncedFlg2/1 -> [VHAL_CAN3BusOff_flg]
  [VHAL_CAN3BusOff_raw] -> DebouncedFlg2/1
  Constant70/1 -> DebouncedFlg2/4
  Constant61/1 -> DebouncedFlg2/3
  Constant60/1 -> DebouncedFlg2/2
  DebouncedFlg3/1 -> [VHAL_CAN4BusOff_flg]
  DebouncedFlg4/1 -> [VHAL_CAN5BusOff_flg]
  DebouncedFlg5/1 -> [VHAL_CAN6BusOff_flg]
  [VHAL_CAN4BusOff_raw] -> DebouncedFlg3/1
  [VHAL_CAN5BusOff_raw] -> DebouncedFlg4/1
  [VHAL_CAN6BusOff_raw] -> DebouncedFlg5/1
  Constant64/1 -> DebouncedFlg3/4
  Constant62/1 -> DebouncedFlg3/2
  Constant63/1 -> DebouncedFlg3/3
  Constant66/1 -> DebouncedFlg4/3
  Constant65/1 -> DebouncedFlg4/2
  Constant67/1 -> DebouncedFlg4/4
  Constant73/1 -> DebouncedFlg5/4
  Constant71/1 -> DebouncedFlg5/2
  Constant72/1 -> DebouncedFlg5/3
  VHAL_CAN1BusOff_raw/1 -> [VHAL_CAN1BusOff_raw]  "VHAL_CAN1BusOff_raw"
  VHAL_CAN1RxErrorCount_raw/1 -> [VHAL_CAN1RxErrorCount_raw]  "VHAL_CAN1RxErrorCount_raw"
  VHAL_CAN1TxErrorCount_raw/1 -> [VHAL_CAN1TxErrorCount_raw]  "VHAL_CAN1TxErrorCount_raw"
  VHAL_CAN2RxErrorCount_raw/1 -> [VHAL_CAN2RxErrorCount_raw]  "VHAL_CAN2RxErrorCount_raw"
  VHAL_CAN2TxErrorCount_raw/1 -> [VHAL_CAN2TxErrorCount_raw]  "VHAL_CAN2TxErrorCount_raw"
  VHAL_CAN3RxErrorCount_raw/1 -> [VHAL_CAN3RxErrorCount_raw]  "VHAL_CAN3RxErrorCount_raw"
  VHAL_CAN3TxErrorCount_raw/1 -> [VHAL_CAN3TxErrorCount_raw]  "VHAL_CAN3TxErrorCount_raw"
  VHAL_CAN4RxErrorCount_raw/1 -> [VHAL_CAN4RxErrorCount_raw]  "VHAL_CAN4RxErrorCount_raw"
  VHAL_CAN4TxErrorCount_raw/1 -> [VHAL_CAN4TxErrorCount_raw]  "VHAL_CAN4TxErrorCount_raw"
  VHAL_CAN5RxErrorCount_raw/1 -> [VHAL_CAN5RxErrorCount_raw]  "VHAL_CAN5RxErrorCount_raw"
  VHAL_CAN5TxErrorCount_raw/1 -> [VHAL_CAN5TxErrorCount_raw]  "VHAL_CAN5TxErrorCount_raw"
  VHAL_CAN6RxErrorCount_raw/1 -> [VHAL_CAN6RxErrorCount_raw]  "VHAL_CAN6RxErrorCount_raw"
  VHAL_CAN6TxErrorCount_raw/1 -> [VHAL_CAN6TxErrorCount_raw]  "VHAL_CAN6TxErrorCount_raw"
  Constant74/1 -> Equal/2
  [VHAL_CAN1RxErrorCount_raw] -> Equal/1
  Equal/1 -> Logical Operator14/1
  Logical Operator14/1 -> [VHAL_CAN1BusError_flg]  "VHAL_CAN1BusError_flg"
  Equal40/1 -> Logical Operator14/2
  [VHAL_CAN1TxErrorCount_raw] -> Equal40/1
  Constant75/1 -> Equal40/2
  Constant77/1 -> Equal42/2
  [VHAL_CAN2TxErrorCount_raw] -> Equal42/1
  Equal42/1 -> Logical Operator15/2
  Logical Operator15/1 -> [VHAL_CAN2BusError_flg]  "VHAL_CAN2BusError_flg"
  Equal41/1 -> Logical Operator15/1
  [VHAL_CAN2RxErrorCount_raw] -> Equal41/1
  Constant76/1 -> Equal41/2
  Constant80/1 -> Equal45/2
  [VHAL_CAN4RxErrorCount_raw] -> Equal45/1
  Equal45/1 -> Logical Operator17/1
  Logical Operator17/1 -> [VHAL_CAN4BusError_flg]  "VHAL_CAN4BusError_flg"
  Equal46/1 -> Logical Operator17/2
  [VHAL_CAN4TxErrorCount_raw] -> Equal46/1
  Constant81/1 -> Equal46/2
  Constant79/1 -> Equal44/2
  [VHAL_CAN3TxErrorCount_raw] -> Equal44/1
  Equal44/1 -> Logical Operator16/2
  Logical Operator16/1 -> [VHAL_CAN3BusError_flg]  "VHAL_CAN3BusError_flg"
  Equal43/1 -> Logical Operator16/1
  [VHAL_CAN3RxErrorCount_raw] -> Equal43/1
  Constant78/1 -> Equal43/2
  Constant82/1 -> Equal47/2
  [VHAL_CAN5RxErrorCount_raw] -> Equal47/1
  Equal47/1 -> Logical Operator18/1
  Logical Operator18/1 -> [VHAL_CAN5BusError_flg]  "VHAL_CAN5BusError_flg"
  Equal48/1 -> Logical Operator18/2
  [VHAL_CAN5TxErrorCount_raw] -> Equal48/1
  Constant83/1 -> Equal48/2
  Constant85/1 -> Equal50/2
  [VHAL_CAN6TxErrorCount_raw] -> Equal50/1
  Equal50/1 -> Logical Operator19/2
  Logical Operator19/1 -> [VHAL_CAN6BusError_flg]  "VHAL_CAN6BusError_flg"
  Equal49/1 -> Logical Operator19/1
  [VHAL_CAN6RxErrorCount_raw] -> Equal49/1
  Constant84/1 -> Equal49/2
  [VHAL_CAN1BusError_flg] -> Bus Creator/246
  [VHAL_CAN2BusError_flg] -> Bus Creator/247
  [VHAL_CAN3BusError_flg] -> Bus Creator/248
  [VHAL_CAN4BusError_flg] -> Bus Creator/249
  [VHAL_CAN5BusError_flg] -> Bus Creator/250
  [VHAL_CAN6BusError_flg] -> Bus Creator/251
  Bus Selector/3 -> [VHAL_DIDGetFoxPiLampCtrl_raw8]  "<VHAL_DIDGetFoxPiLampCtrl_raw8>"
  Bus Selector/4 -> [VHAL_DIDGetFoxPiCtrlEnSw_raw8]  "<VHAL_DIDGetFoxPiCtrlEnSw_raw8>"
  Data Type Conversion113/1 -> [VHAL_RandomnumberY_raw2]  "VHAL_RandomnumberY_raw2"
  Ground9/1 -> Data Type Conversion198/1
  Gain5/1 -> [VHAL_DiagFRTC_mA]  "VHAL_DiagFRTC_mA"
  Ground8/1 -> Data Type Conversion197/1
  Data Type Conversion202/1 -> [VHAL_DiagFMHT_s]  "VHAL_DiagFMHT_s"
  Data Type Conversion115/1 -> [VHAL_RandomnumberY_raw4]  "VHAL_RandomnumberY_raw4"
  Data Type Conversion118/1 -> [VHAL_RandomnumberY_raw7]  "VHAL_RandomnumberY_raw7"
  Demux2/1 -> Data Type Conversion112/1
  Ground13/1 -> [VHAL_APSFunConfig_raw8]
  Demux2/8 -> Data Type Conversion119/1
  Demux2/4 -> Data Type Conversion115/1
  [VHAL_DIDGetDKCKey_raw8] -> Demux2/1
  Data Type Conversion284/1 -> [VHAL_WipRLSCmdHoldEN_flg]  "VHAL_WipRLSCmdHoldEN_flg"
  Data Type Conversion198/1 -> Gain6/1
  Demux2/3 -> Data Type Conversion114/1
  Data Type Conversion112/1 -> [VHAL_RandomnumberY_raw1]  "VHAL_RandomnumberY_raw1"
  Ground4/1 -> Data Type Conversion200/1
  Ground5/1 -> Data Type Conversion201/1
  Data Type Conversion197/1 -> Gain5/1
  Ground3/1 -> Data Type Conversion298/1
  Gain4/1 -> [VHAL_DiagFLTC_mA]  "VHAL_DiagFLTC_mA"
  Data Type Conversion288/1 -> [VHAL_WipRLSCmdCutTime_s]  "VHAL_WipRLSCmdCutTime_s"
  Data Type Conversion201/1 -> [VHAL_DiagDRLOFF_flg]  "VHAL_DiagDRLOFF_flg"
  Data Type Conversion285/1 -> [VHAL_WipRLSCmdHoldTime_s]  "VHAL_WipRLSCmdHoldTime_s"
  Gain6/1 -> [VHAL_DiagRLTC_mA]  "VHAL_DiagRLTC_mA"
  Ground2/1 -> [VHAL_DrivetrainSelect_enum]  "VHAL_DrivetrainSelect_enum"
  Demux2/2 -> Data Type Conversion113/1
  Data Type Conversion114/1 -> [VHAL_RandomnumberY_raw3]  "VHAL_RandomnumberY_raw3"
  Data Type Conversion116/1 -> [VHAL_RandomnumberY_raw5]  "VHAL_RandomnumberY_raw5"
  Data Type Conversion119/1 -> [VHAL_RandomnumberY_raw8]  "VHAL_RandomnumberY_raw8"
  Ground15/1 -> Data Type Conversion283/1
  Ground12/1 -> Data Type Conversion207/1
  Ground14/1 -> [VHAL_FlashRegenMode_enum]
  Data Type Conversion200/1 -> [VHAL_funAuto_flg]  "VHAL_funAuto_flg"
  Data Type Conversion298/1 -> [VHAL_DIDGetDynoMode_flg]  "VHAL_DIDGetDynoMode_flg"
  Data Type Conversion196/1 -> Gain4/1
  Ground17/1 -> Data Type Conversion285/1
  Data Type Conversion117/1 -> [VHAL_RandomnumberY_raw6]  "VHAL_RandomnumberY_raw6"
  Ground10/1 -> Data Type Conversion199/1
  Data Type Conversion207/1 -> [VHAL_TireSize_raw8]
  Demux2/7 -> Data Type Conversion118/1
  Data Type Conversion287/1 -> [VHAL_WipRLSCmdCutEN_flg]  "VHAL_WipRLSCmdCutEN_flg"
  Gain7/1 -> [VHAL_DiagRRTC_mA]  "VHAL_DiagRRTC_mA"
  Demux2/5 -> Data Type Conversion116/1
  Data Type Conversion283/1 -> [VHAL_AutoWipHSpdEN_flg]  "VHAL_AutoWipHSpdEN_flg"
  Ground6/1 -> Data Type Conversion202/1
  Ground7/1 -> Data Type Conversion196/1
  Demux2/6 -> Data Type Conversion117/1
  Data Type Conversion199/1 -> Gain7/1
  Ground11/1 -> [VHAL_USSConfig_raw8]  "VHAL_DrivetrainSelect_enum"
  Ground16/1 -> Data Type Conversion284/1
  Ground18/1 -> Data Type Conversion287/1
  Ground19/1 -> Data Type Conversion288/1
  [BHAL_DIDGetData_raw] -> DIDGet_List/1(BHAL_DIDGetData_raw)
  [VHAL_DIDFlashDKCKey_raw8] -> DIDGet_List/2(VHAL_DIDFlashDKCKey_raw8)
  Ground1/1 -> DIDGet_List/3(VHAL_DIDFlashFoxPiDrivingCtrl_raw8)
  Ground20/1 -> DIDGet_List/4(VHAL_DIDFlashFoxPiLampCtrl_raw8)
  Ground21/1 -> DIDGet_List/5(VHAL_DIDFlashFoxPiCtrlEnSw_raw8)
  DIDGet_List/1(BHAL_DIDOrigOutput_raw8) -> [BHAL_DIDOrigOutput_raw8]
  Bus Selector/2 -> [VHAL_DIDGetFoxPiDrivingCtrl_raw8]  "<VHAL_DIDGetFoxPiDrivingCtrl_raw8>"
  [VHAL_DIDGetFoxPiDrivingCtrl_raw8] -> FoxPiDrivingCtrl/1(VHAL_DIDGetFoxPiDrivingCtrl_raw8)
  FoxPiDrivingCtrl/1(VHAL_FoxPiAccReq_mps2) -> [VHAL_FoxPiAccReq_mps2]
  FoxPiDrivingCtrl/2(VHAL_FoxPiAccReqA_flg) -> [VHAL_FoxPiAccReqA_flg]
  FoxPiDrivingCtrl/3(VHAL_FoxPiTargetSpdReq_kph) -> [VHAL_FoxPiTargetSpdReq_kph]
  FoxPiDrivingCtrl/4(VHAL_FoxPiTargetSpdReqA_flg) -> [VHAL_FoxPiTargetSpdReqA_flg]
  FoxPiDrivingCtrl/5(VHAL_FoxPiAngleTargetValid_flg) -> [VHAL_FoxPiAngleTargetValid_flg]
  FoxPiDrivingCtrl/6(VHAL_FoxPiAngleTargetReq_flg) -> [VHAL_FoxPiAngleTargetReq_flg]
  FoxPiDrivingCtrl/7(VHAL_FoxPiAngleTarget_Deg) -> [VHAL_FoxPiAngleTarget_Deg]
  FoxPiDrivingCtrl/8(VHAL_FoxPiTorqueTargetValid_flg) -> [VHAL_FoxPiTorqueTargetValid_flg]
  FoxPiDrivingCtrl/9(VHAL_FoxPiTorqueTargetReq_flg) -> [VHAL_FoxPiTorqueTargetReq_flg]
  FoxPiDrivingCtrl/10(VHAL_FoxPiTorqueTarget_Nm) -> [VHAL_FoxPiTorqueTarget_Nm]
  FoxPiDrivingCtrl/11(VHAL_FoxPiAPSVMCReqA_flg) -> [VHAL_FoxPiAPSVMCReqA_flg]
  FoxPiDrivingCtrl/12(VHAL_FoxPiAPSStaSystem_enum) -> [VHAL_FoxPiAPSStaSystem_enum]
  FoxPiDrivingCtrl/13(VHAL_FoxPiAPSShiftPosnReq_enum) -> [VHAL_FoxPiAPSShiftPosnReq_enum]
  FoxPiDrivingCtrl/14(VHAL_FoxPiAPSSpeedCMD_kph) -> [VHAL_FoxPiAPSSpeedCMD_kph]
  [VHAL_DIDGetFoxPiCtrlEnSw_raw8] -> Data Type Conversion318/1
  Data Type Conversion318/1 -> [VHAL_FoxPiCtrlEnSw_flg]  "VHAL_FoxPiCtrlEnSw_flg"
  Subsystem/1(VHAL_FoxPiPosLampCtrlEN_flg) -> [VHAL_FoxPiPosLampCtrlEN_flg]
  Subsystem/2(VHAL_FoxPiPosLampCtrl_flg) -> [VHAL_FoxPiPosLampCtrl_flg]
  Subsystem/3(VHAL_FoxPiLBeamCtrlEN_flg) -> [VHAL_FoxPiLBeamCtrlEN_flg]
  Subsystem/4(VHAL_FoxPiLBeamCtrl_flg) -> [VHAL_FoxPiLBeamCtrl_flg]
  Subsystem/5(VHAL_FoxPiHBeamCtrlEN_flg) -> [VHAL_FoxPiHBeamCtrlEN_flg]
  Subsystem/6(VHAL_FoxPiHBeamCtrl_flg) -> [VHAL_FoxPiHBeamCtrl_flg]
  Subsystem/7(VHAL_FoxPiRDRLCtrlEN_flg) -> [VHAL_FoxPiRDRLCtrlEN_flg]
  Subsystem/8(VHAL_FoxPiRDRLCtrl_flg) -> [VHAL_FoxPiRDRLCtrl_flg]
  Subsystem/9(VHAL_FoxPiLDRLCtrlEN_flg) -> [VHAL_FoxPiLDRLCtrlEN_flg]
  Subsystem/10(VHAL_FoxPiLDRLCtrl_flg) -> [VHAL_FoxPiLDRLCtrl_flg]
  Subsystem/11(VHAL_FoxPiLTurnLPCtrlEN_flg) -> [VHAL_FoxPiLTurnLPCtrlEN_flg]
  Subsystem/12(VHAL_FoxPiLTurnLPCtrl_flg) -> [VHAL_FoxPiLTurnLPCtrl_flg]
  Subsystem/13(VHAL_FoxPiRTurnLPCtrlEN_flg) -> [VHAL_FoxPiRTurnLPCtrlEN_flg]
  Subsystem/14(VHAL_FoxPiRTurnLPCtrl_flg) -> [VHAL_FoxPiRTurnLPCtrl_flg]
  Subsystem/15(VHAL_FoxPiBkLampCtrlEN_flg) -> [VHAL_FoxPiBkLampCtrlEN_flg]
  Subsystem/16(VHAL_FoxPiBkLampCtrl_flg) -> [VHAL_FoxPiBkLampCtrl_flg]
  Subsystem/17(VHAL_FoxPiRevCtrlEN_flg) -> [VHAL_FoxPiRevCtrlEN_flg]
  Subsystem/18(VHAL_FoxPiRevCtrl_flg) -> [VHAL_FoxPiRevCtrl_flg]
  Subsystem/19(VHAL_FoxPiRrFogLpCtrlEN_flg) -> [VHAL_FoxPiRrFogLpCtrlEN_flg]
  Subsystem/20(VHAL_FoxPiRrFogLpCtrl_flg) -> [VHAL_FoxPiRrFogLpCtrl_flg]
  Subsystem/21(VHAL_FoxPiAmbCtrlEN_flg) -> [VHAL_FoxPiAmbCtrlEN_flg]
  Subsystem/22(VHAL_FoxPiAmbAreaCtrl_enum) -> [VHAL_FoxPiAmbAreaCtrl_enum]
  Subsystem/23(VHAL_FoxPiAmbColorCtrl_enum) -> [VHAL_FoxPiAmbColorCtrl_enum]
  Subsystem/24(VHAL_FoxPiAmbBrightCtrl_enum) -> [VHAL_FoxPiAmbBrightCtrl_enum]
  Subsystem/25(VHAL_FoxPiAmbBreathCtrl_enum) -> [VHAL_FoxPiAmbBreathCtrl_enum]
  [VHAL_FoxPiCtrlEnSw_flg] -> Bus Creator/252
  [VHAL_FoxPiAccReq_mps2] -> Bus Creator/253
  [VHAL_FoxPiAccReqA_flg] -> Bus Creator/254
  [VHAL_FoxPiTargetSpdReq_kph] -> Bus Creator/255
  [VHAL_FoxPiTargetSpdReqA_flg] -> Bus Creator/256
  [VHAL_FoxPiAngleTargetValid_flg] -> Bus Creator/257
  [VHAL_FoxPiAngleTargetReq_flg] -> Bus Creator/258
  [VHAL_FoxPiAngleTarget_Deg] -> Bus Creator/259
  [VHAL_FoxPiTorqueTargetValid_flg] -> Bus Creator/260
  [VHAL_FoxPiTorqueTargetReq_flg] -> Bus Creator/261
  [VHAL_FoxPiTorqueTarget_Nm] -> Bus Creator/262
  [VHAL_FoxPiAPSVMCReqA_flg] -> Bus Creator/263
  [VHAL_FoxPiAPSStaSystem_enum] -> Bus Creator/264
  [VHAL_FoxPiAPSShiftPosnReq_enum] -> Bus Creator/265
  [VHAL_FoxPiAPSSpeedCMD_kph] -> Bus Creator/266
  [VHAL_FoxPiPosLampCtrlEN_flg] -> Bus Creator/267
  [VHAL_FoxPiPosLampCtrl_flg] -> Bus Creator/268
  [VHAL_FoxPiLBeamCtrlEN_flg] -> Bus Creator/269
  [VHAL_FoxPiLBeamCtrl_flg] -> Bus Creator/270
  [VHAL_FoxPiHBeamCtrlEN_flg] -> Bus Creator/271
  [VHAL_FoxPiHBeamCtrl_flg] -> Bus Creator/272
  [VHAL_FoxPiRDRLCtrlEN_flg] -> Bus Creator/273
  [VHAL_FoxPiRDRLCtrl_flg] -> Bus Creator/274
  [VHAL_FoxPiLDRLCtrlEN_flg] -> Bus Creator/275
  [VHAL_FoxPiLDRLCtrl_flg] -> Bus Creator/276
  [VHAL_FoxPiLTurnLPCtrlEN_flg] -> Bus Creator/277
  [VHAL_FoxPiLTurnLPCtrl_flg] -> Bus Creator/278
  [VHAL_FoxPiRTurnLPCtrlEN_flg] -> Bus Creator/279
  [VHAL_FoxPiRTurnLPCtrl_flg] -> Bus Creator/280
  [VHAL_FoxPiBkLampCtrlEN_flg] -> Bus Creator/281
  [VHAL_FoxPiBkLampCtrl_flg] -> Bus Creator/282
  [VHAL_FoxPiRevCtrlEN_flg] -> Bus Creator/283
  [VHAL_FoxPiRevCtrl_flg] -> Bus Creator/284
  [VHAL_FoxPiRrFogLpCtrlEN_flg] -> Bus Creator/285
  [VHAL_FoxPiRrFogLpCtrl_flg] -> Bus Creator/286
  [VHAL_FoxPiAmbCtrlEN_flg] -> Bus Creator/287
  [VHAL_FoxPiAmbAreaCtrl_enum] -> Bus Creator/288
  [VHAL_FoxPiAmbColorCtrl_enum] -> Bus Creator/289
  [VHAL_FoxPiAmbBrightCtrl_enum] -> Bus Creator/290
  [VHAL_FoxPiAmbBreathCtrl_enum] -> Bus Creator/291
  Constant4/1 -> Equal1/2
  [VHAL_DIDGetFoxPiDrivingCtrl_raw8] -> Equal1/1
  Equal1/1 -> AND/1
  AND/1 -> [VHAL_FoxPiDIDReseted_flg]  "VHAL_FoxPiDIDReseted_flg"
  [VHAL_FoxPiDIDReseted_flg] -> Bus Creator/292
  [VHAL_DIDGetFoxPiLampCtrl_raw8] -> Equal2/1
  Constant1/1 -> Equal2/2
  Switch/1 -> Subsystem/1(VHAL_DIDGetFoxPiLampCtrl_raw8)
  Equal2/1 -> Switch/2
  [VHAL_DIDGetFoxPiLampCtrl_raw8] -> Switch/3
  Constant2/1 -> Switch/1
